simulink model "Ackeraman"  (R2019b)
settings: Solver=VariableStepAuto  StartTime=0.0  StopTime=simTime  RelTol=1e-3
values from neighbouring files (symbols this model uses):
  a0 = 1    [Ackerman_init.m]
  a1 = 4    [Ackerman_init.m]
  a2 = 3    [Ackerman_init.m]
  Change = 0    [Ackerman_init.m]
  k0 = 5    [Ackerman_init.m]
  k1 = place(Ad,bd,pd)    [Ackerman_init.m]
  k2 = place(Ac,bc,lambdatr')    [Ackerman_init.m]
  l = xlabel('Time (s)')    [Ackerman_init.m]
  pathType = 1    [Ackerman_init.m]
  phi0 = 0    [Ackerman_init.m]
  r = 2    [Ackerman_init.m]
  ref0 = [0 0]'    [Ackerman_init.m]
  refType = 1    [Ackerman_init.m]
  T = 0.3    [Ackerman_init.m]
  theta0 = pi    (= 3.14159265359)    [Ackerman_init.m]
  v0 = 2    [Ackerman_init.m]
  v_ref = 2    [Ackerman_init.m]
  x0 = 1    [Ackerman_init.m]
  y0 = 2    [Ackerman_init.m]
libraries: robotmobilelib x4
(part 2 of 4)

== matlab function Ackeraman/MATLAB Function4 ==
  data: state input; v input; v_ref input; c input; pathType parameter; r parameter; a2 parameter; a1 parameter; a0 parameter; k0 parameter; l parameter; u output; w output; Change parameter; T parameter; refType parameter
function [u,w] = MATLAB_Function5(state, v, v_ref, c ,pathType, r, a2, a1, a0, k0, l , Change, T, refType)

x = state(1); y = state(2); z = state(3); theta = state(4);

d = T/3; 
if refType == 1
    L = exp(-k0*T); 
else
    L = 0;  
end
 

if pathType == 1
    w0 = [   -(2*a2*l^2*v^2*cos(theta)^2 - 2*v^3*y*sin(z) - a0*l^2*r^2*cos(theta)^2 - 2*v^3*x*cos(z) + a0*l^2*x^2*cos(theta)^2 + a0*l^2*y^2*cos(theta)^2 + 2*v^3*x*cos(theta)^2*cos(z) + 2*v^3*y*cos(theta)^2*sin(z) + 2*a1*l^2*v*x*cos(theta)^2*cos(z) + 2*a1*l^2*v*y*cos(theta)^2*sin(z) + 2*a2*l*v^2*y*cos(theta)*cos(z)*sin(theta) - 2*a2*l*v^2*x*cos(theta)*sin(theta)*sin(z))/(2*l*v^2*(y*cos(z) - x*sin(z)));
             -(2*a2*l^2*v^2*cos(theta)^2 - 2*v^3*y*sin(z) - a0*l^2*r^2*cos(theta)^2 - 2*v^3*x*cos(z) + a0*l^2*x^2*cos(theta)^2 + a0*l^2*y^2*cos(theta)^2 + 2*v^3*x*cos(theta)^2*cos(z) + 2*v^3*y*cos(theta)^2*sin(z) + 2*a1*l^2*v*x*cos(theta)^2*cos(z) + 2*a1*l^2*v*y*cos(theta)^2*sin(z) + 2*a2*l*v^2*y*cos(theta)*cos(z)*sin(theta) - 2*a2*l*v^2*x*cos(theta)*sin(theta)*sin(z))/(2*l*v^2*(y*cos(z) - x*sin(z)));
             -(2*a2*l^2*v^2*cos(theta)^2 - 2*v^3*y*sin(z) - a0*l^2*r^2*cos(theta)^2 - 2*v^3*x*cos(z) + a0*l^2*x^2*cos(theta)^2 + a0*l^2*y^2*cos(theta)^2 + 2*v^3*x*cos(theta)^2*cos(z) + 2*v^3*y*cos(theta)^2*sin(z) + 2*a1*l^2*v*x*cos(theta)^2*cos(z) + 2*a1*l^2*v*y*cos(theta)^2*sin(z) + 2*a2*l*v^2*y*cos(theta)*cos(z)*sin(theta) - 2*a2*l*v^2*x*cos(theta)*sin(theta)*sin(z))/(2*l*v^2*(y*cos(z) - x*sin(z)))]; 
 
    w1 = [  -(3*(2*l*v^6*y*cos(theta)^3*cos(z) - 2*v^6*y^2*cos(z)^2*sin(theta) - 2*v^6*x^2*sin(theta)*sin(z)^2 - 2*v^6*y^2*sin(theta)*sin(z)^2 - 2*v^6*x^2*cos(z)^2*sin(theta) - 2*l*v^6*x*cos(theta)^3*sin(z) - 2*v^6*x^2*cos(theta)^2*cos(z)^2*sin(theta) + 4*v^6*x^2*cos(theta)^4*cos(z)^2*sin(theta) + 2*v^6*y^2*cos(theta)^2*cos(z)^2*sin(theta) + 2*v^6*x^2*cos(theta)^2*sin(theta)*sin(z)^2 - 2*v^6*y^2*cos(theta)^2*sin(theta)*sin(z)^2 + 4*v^6*y^2*cos(theta)^4*sin(theta)*sin(z)^2 - 2*l*v^6*y*cos(theta)*cos(z) + a0^2*l^4*r^4*cos(theta)^4*sin(theta) + 2*l*v^6*x*cos(theta)*sin(z) + 4*a2^2*l^4*v^4*cos(theta)^4*sin(theta) + a0^2*l^4*x^4*cos(theta)^4*sin(theta) + a0^2*l^4*y^4*cos(theta)^4*sin(theta) - 2*a2^2*l^3*v^4*y*cos(theta)^3*cos(z) + 2*a2^2*l^3*v^4*x*cos(theta)^3*sin(z) - 2*a0^2*l^4*r^2*x^2*cos(theta)^4*sin(theta) - 2*a0^2*l^4*r^2*y^2*cos(theta)^4*sin(theta) + 2*a0^2*l^4*x^2*y^2*cos(theta)^4*sin(theta) + 2*a1*l^3*v^4*y*cos(theta)^3*cos(z) - 2*a1*l^3*v^4*x*cos(theta)^3*sin(z) - 2*a2^2*l^2*v^4*x^2*cos(theta)^2*sin(theta)*sin(z)^2 + 4*a1^2*l^4*v^2*y^2*cos(theta)^4*sin(theta)*sin(z)^2 - 8*v^6*x*y*cos(theta)^2*cos(z)*sin(theta)*sin(z) + 8*v^6*x*y*cos(theta)^4*cos(z)*sin(theta)*sin(z) - a0*l^2*v^3*x^3*cos(theta)^2*cos(z)*sin(theta) + 4*a0*l^2*v^3*x^3*cos(theta)^4*cos(z)*sin(theta) - 2*a0*l^3*v^3*x^2*cos(theta)^3*cos(z)*sin(z) + 2*a0*l^3*v^3*y^2*cos(theta)^3*cos(z)*sin(z) - a0*l^2*v^3*y^3*cos(theta)^2*sin(theta)*sin(z) + 4*a0*l^2*v^3*y^3*cos(theta)^4*sin(theta)*sin(z) + 4*a2^2*l^2*v^4*y^2*cos(theta)^2*cos(z)^2*sin(theta)^3 + 4*a2^2*l^2*v^4*x^2*cos(theta)^2*sin(theta)^3*sin(z)^2 - 2*a1*l^2*v^4*x^2*cos(theta)^2*cos(z)^2*sin(theta) + 8*a1*l^2*v^4*x^2*cos(theta)^4*cos(z)^2*sin(theta) + 2*a1*l^2*v^4*y^2*cos(theta)^2*cos(z)^2*sin(theta) + 8*a2^2*l^3*v^4*y*cos(theta)^3*cos(z)*sin(theta)^2 + 2*a1*l^2*v^4*x^2*cos(theta)^2*sin(theta)*sin(z)^2 - 8*a2^2*l^3*v^4*x*cos(theta)^3*sin(theta)^2*sin(z) - 2*a1*l^2*v^4*y^2*cos(theta)^2*sin(theta)*sin(z)^2 + 8*a1*l^2*v^4*y^2*cos(theta)^4*sin(theta)*sin(z)^2 - a0*a2*l^3*v^2*y^3*cos(theta)^3*cos(z) - 4*a0*a2*l^4*r^2*v^2*cos(theta)^4*sin(theta) + 4*a0*a2*l^4*v^2*x^2*cos(theta)^4*sin(theta) + 4*a0*a2*l^4*v^2*y^2*cos(theta)^4*sin(theta) + a0*a2*l^3*v^2*x^3*cos(theta)^3*sin(z) + 2*a0*l^3*v^3*x*y*cos(theta)^3*cos(z)^2 - 2*a2*l^2*v^5*x*cos(theta)^2*cos(z)*sin(theta) + 8*a2*l^2*v^5*x*cos(theta)^4*cos(z)*sin(theta) - 2*a0*l^3*v^3*x*y*cos(theta)^3*sin(z)^2 - 2*a2*l^2*v^5*y*cos(theta)^2*sin(theta)*sin(z) + 8*a2*l^2*v^5*y*cos(theta)^4*sin(theta)*sin(z) + 4*a1^2*l^4*v^2*x^2*cos(theta)^4*cos(z)^2*sin(theta) - 2*a2^2*l^2*v^4*y^2*cos(theta)^2*cos(z)^2*sin(theta) - 4*a0*a2*l^3*v^2*x^3*cos(theta)^3*sin(theta)^2*sin(z) + a0*a2*l^3*r^2*v^2*y*cos(theta)^3*cos(z) - 8*a2*l*v^5*x^2*cos(theta)^3*cos(z)*sin(theta)^2*sin(z) + 8*a2*l*v^5*y^2*cos(theta)^3*cos(z)*sin(theta)^2*sin(z) - a0*a2*l^3*v^2*x^2*y*cos(theta)^3*cos(z) - 2*a1*a2*l^3*v^3*x*y*cos(theta)^3*cos(z)^2 - a0*a2*l^3*r^2*v^2*x*cos(theta)^3*sin(z) + 4*a0*a1*l^4*v*x^3*cos(theta)^4*cos(z)*sin(theta) + 8*a1*a2*l^4*v^3*x*cos(theta)^4*cos(z)*sin(theta) + a0*a2*l^3*v^2*x*y^2*cos(theta)^3*sin(z) + 2*a1*a2*l^3*v^3*x*y*cos(theta)^3*sin(z)^2 + 4*a0*a1*l^4*v*y^3*cos(theta)^4*sin(theta)*sin(z) + 8*a1*a2*l^4*v^3*y*cos(theta)^4*sin(theta)*sin(z) - 2*a2*l*v^5*x*y*cos(theta)*cos(z)^2*sin(theta)^2 + 2*a2*l*v^5*x*y*cos(theta)*sin(theta)^2*sin(z)^2 + 2*a1*a2*l^3*v^3*x^2*cos(theta)^3*cos(z)*sin(z) - 2*a1*a2*l^3*v^3*y^2*cos(theta)^3*cos(z)*sin(z) + a0*l^2*r^2*v^3*x*cos(theta)^2*cos(z)*sin(theta) - 4*a0*l^2*r^2*v^3*x*cos(theta)^4*cos(z)*sin(theta) - a0*l^2*v^3*x*y^2*cos(theta)^2*cos(z)*sin(theta) + 4*a0*l^2*v^3*x*y^2*cos(theta)^4*cos(z)*sin(theta) + 8*a2*l*v^5*x*y*cos(theta)^3*cos(z)^2*sin(theta)^2 + a0*l^2*r^2*v^3*y*cos(theta)^2*sin(theta)*sin(z) - 4*a0*l^2*r^2*v^3*y*cos(theta)^4*sin(theta)*sin(z) - a0*l^2*v^3*x^2*y*cos(theta)^2*sin(theta)*sin(z) + 4*a0*l^2*v^3*x^2*y*cos(theta)^4*sin(theta)*sin(z) - 8*a2*l*v^5*x*y*cos(theta)^3*sin(theta)^2*sin(z)^2 + 2*a2*l*v^5*x^2*cos(theta)*cos(z)*sin(theta)^2*sin(z) - 2*a2*l*v^5*y^2*cos(theta)*cos(z)*sin(theta)^2*sin(z) + 4*a0*a2*l^3*v^2*y^3*cos(theta)^3*cos(z)*sin(theta)^2 - 8*a1*l^2*v^4*x*y*cos(theta)^2*cos(z)*sin(theta)*sin(z) + 16*a1*l^2*v^4*x*y*cos(theta)^4*cos(z)*sin(theta)*sin(z) - 4*a0*a2*l^3*r^2*v^2*y*cos(theta)^3*cos(z)*sin(theta)^2 + 4*a0*a2*l^3*v^2*x^2*y*cos(theta)^3*cos(z)*sin(theta)^2 + 8*a1*a2*l^3*v^3*x*y*cos(theta)^3*cos(z)^2*sin(theta)^2 + 4*a0*a2*l^3*r^2*v^2*x*cos(theta)^3*sin(theta)^2*sin(z) - 4*a0*a2*l^3*v^2*x*y^2*cos(theta)^3*sin(theta)^2*sin(z) - 8*a1*a2*l^3*v^3*x*y*cos(theta)^3*sin(theta)^2*sin(z)^2 + 4*a2^2*l^2*v^4*x*y*cos(theta)^2*cos(z)*sin(theta)*sin(z) + 8*a1^2*l^4*v^2*x*y*cos(theta)^4*cos(z)*sin(theta)*sin(z) - 4*a0*a1*l^4*r^2*v*x*cos(theta)^4*cos(z)*sin(theta) + 4*a0*a1*l^4*v*x*y^2*cos(theta)^4*cos(z)*sin(theta) - 4*a0*a1*l^4*r^2*v*y*cos(theta)^4*sin(theta)*sin(z) + 4*a0*a1*l^4*v*x^2*y*cos(theta)^4*sin(theta)*sin(z) - 8*a1*a2*l^3*v^3*x^2*cos(theta)^3*cos(z)*sin(theta)^2*sin(z) + 8*a1*a2*l^3*v^3*y^2*cos(theta)^3*cos(z)*sin(theta)^2*sin(z) - 8*a2^2*l^2*v^4*x*y*cos(theta)^2*cos(z)*sin(theta)^3*sin(z)))/(8*l^2*v^4*cos(theta)*(y*cos(z) - x*sin(z))^2);
            -(3*(2*l*v^6*y*cos(theta)^3*cos(z) - 2*v^6*y^2*cos(z)^2*sin(theta) - 2*v^6*x^2*sin(theta)*sin(z)^2 - 2*v^6*y^2*sin(theta)*sin(z)^2 - 2*v^6*x^2*cos(z)^2*sin(theta) - 2*l*v^6*x*cos(theta)^3*sin(z) - 2*v^6*x^2*cos(theta)^2*cos(z)^2*sin(theta) + 4*v^6*x^2*cos(theta)^4*cos(z)^2*sin(theta) + 2*v^6*y^2*cos(theta)^2*cos(z)^2*sin(theta) + 2*v^6*x^2*cos(theta)^2*sin(theta)*sin(z)^2 - 2*v^6*y^2*cos(theta)^2*sin(theta)*sin(z)^2 + 4*v^6*y^2*cos(theta)^4*sin(theta)*sin(z)^2 - 2*l*v^6*y*cos(theta)*cos(z) + a0^2*l^4*r^4*cos(theta)^4*sin(theta) + 2*l*v^6*x*cos(theta)*sin(z) + 4*a2^2*l^4*v^4*cos(theta)^4*sin(theta) + a0^2*l^4*x^4*cos(theta)^4*sin(theta) + a0^2*l^4*y^4*cos(theta)^4*sin(theta) - 2*a2^2*l^3*v^4*y*cos(theta)^3*cos(z) + 2*a2^2*l^3*v^4*x*cos(theta)^3*sin(z) - 2*a0^2*l^4*r^2*x^2*cos(theta)^4*sin(theta) - 2*a0^2*l^4*r^2*y^2*cos(theta)^4*sin(theta) + 2*a0^2*l^4*x^2*y^2*cos(theta)^4*sin(theta) + 2*a1*l^3*v^4*y*cos(theta)^3*cos(z) - 2*a1*l^3*v^4*x*cos(theta)^3*sin(z) - 2*a2^2*l^2*v^4*x^2*cos(theta)^2*sin(theta)*sin(z)^2 + 4*a1^2*l^4*v^2*y^2*cos(theta)^4*sin(theta)*sin(z)^2 - 8*v^6*x*y*cos(theta)^2*cos(z)*sin(theta)*sin(z) + 8*v^6*x*y*cos(theta)^4*cos(z)*sin(theta)*sin(z) - a0*l^2*v^3*x^3*cos(theta)^2*cos(z)*sin(theta) + 4*a0*l^2*v^3*x^3*cos(theta)^4*cos(z)*sin(theta) - 2*a0*l^3*v^3*x^2*cos(theta)^3*cos(z)*sin(z) + 2*a0*l^3*v^3*y^2*cos(theta)^3*cos(z)*sin(z) - a0*l^2*v^3*y^3*cos(theta)^2*sin(theta)*sin(z) + 4*a0*l^2*v^3*y^3*cos(theta)^4*sin(theta)*sin(z) + 4*a2^2*l^2*v^4*y^2*cos(theta)^2*cos(z)^2*sin(theta)^3 + 4*a2^2*l^2*v^4*x^2*cos(theta)^2*sin(theta)^3*sin(z)^2 - 2*a1*l^2*v^4*x^2*cos(theta)^2*cos(z)^2*sin(theta) + 8*a1*l^2*v^4*x^2*cos(theta)^4*cos(z)^2*sin(theta) + 2*a1*l^2*v^4*y^2*cos(theta)^2*cos(z)^2*sin(theta) + 8*a2^2*l^3*v^4*y*cos(theta)^3*cos(z)*sin(theta)^2 + 2*a1*l^2*v^4*x^2*cos(theta)^2*sin(theta)*sin(z)^2 - 8*a2^2*l^3*v^4*x*cos(theta)^3*sin(theta)^2*sin(z) - 2*a1*l^2*v^4*y^2*cos(theta)^2*sin(theta)*sin(z)^2 + 8*a1*l^2*v^4*y^2*cos(theta)^4*sin(theta)*sin(z)^2 - a0*a2*l^3*v^2*y^3*cos(theta)^3*cos(z) - 4*a0*a2*l^4*r^2*v^2*cos(theta)^4*sin(theta) + 4*a0*a2*l^4*v^2*x^2*cos(theta)^4*sin(theta) + 4*a0*a2*l^4*v^2*y^2*cos(theta)^4*sin(theta) + a0*a2*l^3*v^2*x^3*cos(theta)^3*sin(z) + 2*a0*l^3*v^3*x*y*cos(theta)^3*cos(z)^2 - 2*a2*l^2*v^5*x*cos(theta)^2*cos(z)*sin(theta) + 8*a2*l^2*v^5*x*cos(theta)^4*cos(z)*sin(theta) - 2*a0*l^3*v^3*x*y*cos(theta)^3*sin(z)^2 - 2*a2*l^2*v^5*y*cos(theta)^2*sin(theta)*sin(z) + 8*a2*l^2*v^5*y*cos(theta)^4*sin(theta)*sin(z) + 4*a1^2*l^4*v^2*x^2*cos(theta)^4*cos(z)^2*sin(theta) - 2*a2^2*l^2*v^4*y^2*cos(theta)^2*cos(z)^2*sin(theta) - 4*a0*a2*l^3*v^2*x^3*cos(theta)^3*sin(theta)^2*sin(z) + a0*a2*l^3*r^2*v^2*y*cos(theta)^3*cos(z) - 8*a2*l*v^5*x^2*cos(theta)^3*cos(z)*sin(theta)^2*sin(z) + 8*a2*l*v^5*y^2*cos(theta)^3*cos(z)*sin(theta)^2*sin(z) - a0*a2*l^3*v^2*x^2*y*cos(theta)^3*cos(z) - 2*a1*a2*l^3*v^3*x*y*cos(theta)^3*cos(z)^2 - a0*a2*l^3*r^2*v^2*x*cos(theta)^3*sin(z) + 4*a0*a1*l^4*v*x^3*cos(theta)^4*cos(z)*sin(theta) + 8*a1*a2*l^4*v^3*x*cos(theta)^4*cos(z)*sin(theta) + a0*a2*l^3*v^2*x*y^2*cos(theta)^3*sin(z) + 2*a1*a2*l^3*v^3*x*y*cos(theta)^3*sin(z)^2 + 4*a0*a1*l^4*v*y^3*cos(theta)^4*sin(theta)*sin(z) + 8*a1*a2*l^4*v^3*y*cos(theta)^4*sin(theta)*sin(z) - 2*a2*l*v^5*x*y*cos(theta)*cos(z)^2*sin(theta)^2 + 2*a2*l*v^5*x*y*cos(theta)*sin(theta)^2*sin(z)^2 + 2*a1*a2*l^3*v^3*x^2*cos(theta)^3*cos(z)*sin(z) - 2*a1*a2*l^3*v^3*y^2*cos(theta)^3*cos(z)*sin(z) + a0*l^2*r^2*v^3*x*cos(theta)^2*cos(z)*sin(theta) - 4*a0*l^2*r^2*v^3*x*cos(theta)^4*cos(z)*sin(theta) - a0*l^2*v^3*x*y^2*cos(theta)^2*cos(z)*sin(theta) + 4*a0*l^2*v^3*x*y^2*cos(theta)^4*cos(z)*sin(theta) + 8*a2*l*v^5*x*y*cos(theta)^3*cos(z)^2*sin(theta)^2 + a0*l^2*r^2*v^3*y*cos(theta)^2*sin(theta)*sin(z) - 4*a0*l^2*r^2*v^3*y*cos(theta)^4*sin(theta)*sin(z) - a0*l^2*v^3*x^2*y*cos(theta)^2*sin(theta)*sin(z) + 4*a0*l^2*v^3*x^2*y*cos(theta)^4*sin(theta)*sin(z) - 8*a2*l*v^5*x*y*cos(theta)^3*sin(theta)^2*sin(z)^2 + 2*a2*l*v^5*x^2*cos(theta)*cos(z)*sin(theta)^2*sin(z) - 2*a2*l*v^5*y^2*cos(theta)*cos(z)*sin(theta)^2*sin(z) + 4*a0*a2*l^3*v^2*y^3*cos(theta)^3*cos(z)*sin(theta)^2 - 8*a1*l^2*v^4*x*y*cos(theta)^2*cos(z)*sin(theta)*sin(z) + 16*a1*l^2*v^4*x*y*cos(theta)^4*cos(z)*sin(theta)*sin(z) - 4*a0*a2*l^3*r^2*v^2*y*cos(theta)^3*cos(z)*sin(theta)^2 + 4*a0*a2*l^3*v^2*x^2*y*cos(theta)^3*cos(z)*sin(theta)^2 + 8*a1*a2*l^3*v^3*x*y*cos(theta)^3*cos(z)^2*sin(theta)^2 + 4*a0*a2*l^3*r^2*v^2*x*cos(theta)^3*sin(theta)^2*sin(z) - 4*a0*a2*l^3*v^2*x*y^2*cos(theta)^3*sin(theta)^2*sin(z) - 8*a1*a2*l^3*v^3*x*y*cos(theta)^3*sin(theta)^2*sin(z)^2 + 4*a2^2*l^2*v^4*x*y*cos(theta)^2*cos(z)*sin(theta)*sin(z) + 8*a1^2*l^4*v^2*x*y*cos(theta)^4*cos(z)*sin(theta)*sin(z) - 4*a0*a1*l^4*r^2*v*x*cos(theta)^4*cos(z)*sin(theta) + 4*a0*a1*l^4*v*x*y^2*cos(theta)^4*cos(z)*sin(theta) - 4*a0*a1*l^4*r^2*v*y*cos(theta)^4*sin(theta)*sin(z) + 4*a0*a1*l^4*v*x^2*y*cos(theta)^4*sin(theta)*sin(z) - 8*a1*a2*l^3*v^3*x^2*cos(theta)^3*cos(z)*sin(theta)^2*sin(z) + 8*a1*a2*l^3*v^3*y^2*cos(theta)^3*cos(z)*sin(theta)^2*sin(z) - 8*a2^2*l^2*v^4*x*y*cos(theta)^2*cos(z)*sin(theta)^3*sin(z)))/(2*l^2*v^4*cos(theta)*(y*cos(z) - x*sin(z))^2);
            -(21*(2*l*v^6*y*cos(theta)^3*cos(z) - 2*v^6*y^2*cos(z)^2*sin(theta) - 2*v^6*x^2*sin(theta)*sin(z)^2 - 2*v^6*y^2*sin(theta)*sin(z)^2 - 2*v^6*x^2*cos(z)^2*sin(theta) - 2*l*v^6*x*cos(theta)^3*sin(z) - 2*v^6*x^2*cos(theta)^2*cos(z)^2*sin(theta) + 4*v^6*x^2*cos(theta)^4*cos(z)^2*sin(theta) + 2*v^6*y^2*cos(theta)^2*cos(z)^2*sin(theta) + 2*v^6*x^2*cos(theta)^2*sin(theta)*sin(z)^2 - 2*v^6*y^2*cos(theta)^2*sin(theta)*sin(z)^2 + 4*v^6*y^2*cos(theta)^4*sin(theta)*sin(z)^2 - 2*l*v^6*y*cos(theta)*cos(z) + a0^2*l^4*r^4*cos(theta)^4*sin(theta) + 2*l*v^6*x*cos(theta)*sin(z) + 4*a2^2*l^4*v^4*cos(theta)^4*sin(theta) + a0^2*l^4*x^4*cos(theta)^4*sin(theta) + a0^2*l^4*y^4*cos(theta)^4*sin(theta) - 2*a2^2*l^3*v^4*y*cos(theta)^3*cos(z) + 2*a2^2*l^3*v^4*x*cos(theta)^3*sin(z) - 2*a0^2*l^4*r^2*x^2*cos(theta)^4*sin(theta) - 2*a0^2*l^4*r^2*y^2*cos(theta)^4*sin(theta) + 2*a0^2*l^4*x^2*y^2*cos(theta)^4*sin(theta) + 2*a1*l^3*v^4*y*cos(theta)^3*cos(z) - 2*a1*l^3*v^4*x*cos(theta)^3*sin(z) - 2*a2^2*l^2*v^4*x^2*cos(theta)^2*sin(theta)*sin(z)^2 + 4*a1^2*l^4*v^2*y^2*cos(theta)^4*sin(theta)*sin(z)^2 - 8*v^6*x*y*cos(theta)^2*cos(z)*sin(theta)*sin(z) + 8*v^6*x*y*cos(theta)^4*cos(z)*sin(theta)*sin(z) - a0*l^2*v^3*x^3*cos(theta)^2*cos(z)*sin(theta) + 4*a0*l^2*v^3*x^3*cos(theta)^4*cos(z)*sin(theta) - 2*a0*l^3*v^3*x^2*cos(theta)^3*cos(z)*sin(z) + 2*a0*l^3*v^3*y^2*cos(theta)^3*cos(z)*sin(z) - a0*l^2*v^3*y^3*cos(theta)^2*sin(theta)*sin(z) + 4*a0*l^2*v^3*y^3*cos(theta)^4*sin(theta)*sin(z) + 4*a2^2*l^2*v^4*y^2*cos(theta)^2*cos(z)^2*sin(theta)^3 + 4*a2^2*l^2*v^4*x^2*cos(theta)^2*sin(theta)^3*sin(z)^2 - 2*a1*l^2*v^4*x^2*cos(theta)^2*cos(z)^2*sin(theta) + 8*a1*l^2*v^4*x^2*cos(theta)^4*cos(z)^2*sin(theta) + 2*a1*l^2*v^4*y^2*cos(theta)^2*cos(z)^2*sin(theta) + 8*a2^2*l^3*v^4*y*cos(theta)^3*cos(z)*sin(theta)^2 + 2*a1*l^2*v^4*x^2*cos(theta)^2*sin(theta)*sin(z)^2 - 8*a2^2*l^3*v^4*x*cos(theta)^3*sin(theta)^2*sin(z) - 2*a1*l^2*v^4*y^2*cos(theta)^2*sin(theta)*sin(z)^2 + 8*a1*l^2*v^4*y^2*cos(theta)^4*sin(theta)*sin(z)^2 - a0*a2*l^3*v^2*y^3*cos(theta)^3*cos(z) - 4*a0*a2*l^4*r^2*v^2*cos(theta)^4*sin(theta) + 4*a0*a2*l^4*v^2*x^2*cos(theta)^4*sin(theta) + 4*a0*a2*l^4*v^2*y^2*cos(theta)^4*sin(theta) + a0*a2*l^3*v^2*x^3*cos(theta)^3*sin(z) + 2*a0*l^3*v^3*x*y*cos(theta)^3*cos(z)^2 - 2*a2*l^2*v^5*x*cos(theta)^2*cos(z)*sin(theta) + 8*a2*l^2*v^5*x*cos(theta)^4*cos(z)*sin(theta) - 2*a0*l^3*v^3*x*y*cos(theta)^3*sin(z)^2 - 2*a2*l^2*v^5*y*cos(theta)^2*sin(theta)*sin(z) + 8*a2*l^2*v^5*y*cos(theta)^4*sin(theta)*sin(z) + 4*a1^2*l^4*v^2*x^2*cos(theta)^4*cos(z)^2*sin(theta) - 2*a2^2*l^2*v^4*y^2*cos(theta)^2*cos(z)^2*sin(theta) - 4*a0*a2*l^3*v^2*x^3*cos(theta)^3*sin(theta)^2*sin(z) + a0*a2*l^3*r^2*v^2*y*cos(theta)^3*cos(z) - 8*a2*l*v^5*x^2*cos(theta)^3*cos(z)*sin(theta)^2*sin(z) + 8*a2*l*v^5*y^2*cos(theta)^3*cos(z)*sin(theta)^2*sin(z) - a0*a2*l^3*v^2*x^2*y*cos(theta)^3*cos(z) - 2*a1*a2*l^3*v^3*x*y*cos(theta)^3*cos(z)^2 - a0*a2*l^3*r^2*v^2*x*cos(theta)^3*sin(z) + 4*a0*a1*l^4*v*x^3*cos(theta)^4*cos(z)*sin(theta) + 8*a1*a2*l^4*v^3*x*cos(theta)^4*cos(z)*sin(theta) + a0*a2*l^3*v^2*x*y^2*cos(theta)^3*sin(z) + 2*a1*a2*l^3*v^3*x*y*cos(theta)^3*sin(z)^2 + 4*a0*a1*l^4*v*y^3*cos(theta)^4*sin(theta)*sin(z) + 8*a1*a2*l^4*v^3*y*cos(theta)^4*sin(theta)*sin(z) - 2*a2*l*v^5*x*y*cos(theta)*cos(z)^2*sin(theta)^2 + 2*a2*l*v^5*x*y*cos(theta)*sin(theta)^2*sin(z)^2 + 2*a1*a2*l^3*v^3*x^2*cos(theta)^3*cos(z)*sin(z) - 2*a1*a2*l^3*v^3*y^2*cos(theta)^3*cos(z)*sin(z) + a0*l^2*r^2*v^3*x*cos(theta)^2*cos(z)*sin(theta) - 4*a0*l^2*r^2*v^3*x*cos(theta)^4*cos(z)*sin(theta) - a0*l^2*v^3*x*y^2*cos(theta)^2*cos(z)*sin(theta) + 4*a0*l^2*v^3*x*y^2*cos(theta)^4*cos(z)*sin(theta) + 8*a2*l*v^5*x*y*cos(theta)^3*cos(z)^2*sin(theta)^2 + a0*l^2*r^2*v^3*y*cos(theta)^2*sin(theta)*sin(z) - 4*a0*l^2*r^2*v^3*y*cos(theta)^4*sin(theta)*sin(z) - a0*l^2*v^3*x^2*y*cos(theta)^2*sin(theta)*sin(z) + 4*a0*l^2*v^3*x^2*y*cos(theta)^4*sin(theta)*sin(z) - 8*a2*l*v^5*x*y*cos(theta)^3*sin(theta)^2*sin(z)^2 + 2*a2*l*v^5*x^2*cos(theta)*cos(z)*sin(theta)^2*sin(z) - 2*a2*l*v^5*y^2*cos(theta)*cos(z)*sin(theta)^2*sin(z) + 4*a0*a2*l^3*v^2*y^3*cos(theta)^3*cos(z)*sin(theta)^2 - 8*a1*l^2*v^4*x*y*cos(theta)^2*cos(z)*sin(theta)*sin(z) + 16*a1*l^2*v^4*x*y*cos(theta)^4*cos(z)*sin(theta)*sin(z) - 4*a0*a2*l^3*r^2*v^2*y*cos(theta)^3*cos(z)*sin(theta)^2 + 4*a0*a2*l^3*v^2*x^2*y*cos(theta)^3*cos(z)*sin(theta)^2 + 8*a1*a2*l^3*v^3*x*y*cos(theta)^3*cos(z)^2*sin(theta)^2 + 4*a0*a2*l^3*r^2*v^2*x*cos(theta)^3*sin(theta)^2*sin(z) - 4*a0*a2*l^3*v^2*x*y^2*cos(theta)^3*sin(theta)^2*sin(z) - 8*a1*a2*l^3*v^3*x*y*cos(theta)^3*sin(theta)^2*sin(z)^2 + 4*a2^2*l^2*v^4*x*y*cos(theta)^2*cos(z)*sin(theta)*sin(z) + 8*a1^2*l^4*v^2*x*y*cos(theta)^4*cos(z)*sin(theta)*sin(z) - 4*a0*a1*l^4*r^2*v*x*cos(theta)^4*cos(z)*sin(theta) + 4*a0*a1*l^4*v*x*y^2*cos(theta)^4*cos(z)*sin(theta) - 4*a0*a1*l^4*r^2*v*y*cos(theta)^4*sin(theta)*sin(z) + 4*a0*a1*l^4*v*x^2*y*cos(theta)^4*sin(theta)*sin(z) - 8*a1*a2*l^3*v^3*x^2*cos(theta)^3*cos(z)*sin(theta)^2*sin(z) + 8*a1*a2*l^3*v^3*y^2*cos(theta)^3*cos(z)*sin(theta)^2*sin(z) - 8*a2^2*l^2*v^4*x*y*cos(theta)^2*cos(z)*sin(theta)^3*sin(z)))/(8*l^2*v^4*cos(theta)*(y*cos(z) - x*sin(z))^2)];

else
    
       w0 = [-(2533274790395904*v^3*x*cos(z) - 2533274790395904*v^3*y*sin(z) - 1228357238169957*a0*l^2*cos(theta)^2 - 281474976710656*v^3*x^3*cos(z) - 281474976710656*v^3*y^3*sin(z) + 281474976710656*v^3*x^3*cos(theta)^2*cos(z) + 281474976710656*v^3*y^3*cos(theta)^2*sin(z) - 281474976710656*v^3*x*y^2*cos(z) - 281474976710656*v^3*x^2*y*sin(z) + 2533274790395904*a2*l^2*v^2*cos(theta)^2 - 1266637395197952*a0*l^2*x^2*cos(theta)^2 + 70368744177664*a0*l^2*x^4*cos(theta)^2 + 1266637395197952*a0*l^2*y^2*cos(theta)^2 + 70368744177664*a0*l^2*y^4*cos(theta)^2 - 2533274790395904*v^3*x*cos(theta)^2*cos(z) + 2533274790395904*v^3*y*cos(theta)^2*sin(z) + 281474976710656*a2*l^2*v^2*x^2*cos(theta)^2 + 844424930131968*a2*l^2*v^2*y^2*cos(theta)^2 + 140737488355328*a0*l^2*x^2*y^2*cos(theta)^2 + 1688849860263936*l^2*v^3*x*cos(theta)^2*cos(z) + 281474976710656*v^3*x*y^2*cos(theta)^2*cos(z) + 1688849860263936*l^2*v^3*y*cos(theta)^2*sin(z) + 281474976710656*v^3*x^2*y*cos(theta)^2*sin(z) - 5066549580791808*a2*l^2*v^2*cos(theta)^2*cos(z)^2 - 844424930131968*l*v^3*x*y*sin(2*theta) + 15199648742375424*l*v^3*cos(theta)*cos(z)*sin(theta)*sin(z) - 2533274790395904*a1*l^2*v*x*cos(theta)^2*cos(z) + 2533274790395904*a1*l^2*v*y*cos(theta)^2*sin(z) + 562949953421312*a2*l^2*v^2*x^2*cos(theta)^2*cos(z)^2 - 562949953421312*a2*l^2*v^2*y^2*cos(theta)^2*cos(z)^2 + 281474976710656*a1*l^2*v*x^3*cos(theta)^2*cos(z) + 281474976710656*a1*l^2*v*y^3*cos(theta)^2*sin(z) - 1688849860263936*l*v^3*x^2*cos(theta)*cos(z)*sin(theta)*sin(z) + 1688849860263936*l*v^3*y^2*cos(theta)*cos(z)*sin(theta)*sin(z) + 2533274790395904*a2*l*v^2*y*cos(theta)*cos(z)*sin(theta) + 2533274790395904*a2*l*v^2*x*cos(theta)*sin(theta)*sin(z) + 281474976710656*a1*l^2*v*x*y^2*cos(theta)^2*cos(z) + 281474976710656*a1*l^2*v*x^2*y*cos(theta)^2*sin(z) + 281474976710656*a2*l*v^2*y^3*cos(theta)*cos(z)*sin(theta) - 281474976710656*a2*l*v^2*x^3*cos(theta)*sin(theta)*sin(z) + 3377699720527872*l*v^3*x*y*cos(theta)*cos(z)^2*sin(theta) + 1125899906842624*a2*l^2*v^2*x*y*cos(theta)^2*cos(z)*sin(z) + 281474976710656*a2*l*v^2*x^2*y*cos(theta)*cos(z)*sin(theta) - 281474976710656*a2*l*v^2*x*y^2*cos(theta)*sin(theta)*sin(z))/(281474976710656*l*v^2*(- sin(z)*x^3 + cos(z)*x^2*y - sin(z)*x*y^2 + 9*sin(z)*x + cos(z)*y^3 + 9*cos(z)*y));
        -(2533274790395904*v^3*x*cos(z) - 2533274790395904*v^3*y*sin(z) - 1228357238169957*a0*l^2*cos(theta)^2 - 281474976710656*v^3*x^3*cos(z) - 281474976710656*v^3*y^3*sin(z) + 281474976710656*v^3*x^3*cos(theta)^2*cos(z) + 281474976710656*v^3*y^3*cos(theta)^2*sin(z) - 281474976710656*v^3*x*y^2*cos(z) - 281474976710656*v^3*x^2*y*sin(z) + 2533274790395904*a2*l^2*v^2*cos(theta)^2 - 1266637395197952*a0*l^2*x^2*cos(theta)^2 + 70368744177664*a0*l^2*x^4*cos(theta)^2 + 1266637395197952*a0*l^2*y^2*cos(theta)^2 + 70368744177664*a0*l^2*y^4*cos(theta)^2 - 2533274790395904*v^3*x*cos(theta)^2*cos(z) + 2533274790395904*v^3*y*cos(theta)^2*sin(z) + 281474976710656*a2*l^2*v^2*x^2*cos(theta)^2 + 844424930131968*a2*l^2*v^2*y^2*cos(theta)^2 + 140737488355328*a0*l^2*x^2*y^2*cos(theta)^2 + 1688849860263936*l^2*v^3*x*cos(theta)^2*cos(z) + 281474976710656*v^3*x*y^2*cos(theta)^2*cos(z) + 1688849860263936*l^2*v^3*y*cos(theta)^2*sin(z) + 281474976710656*v^3*x^2*y*cos(theta)^2*sin(z) - 5066549580791808*a2*l^2*v^2*cos(theta)^2*cos(z)^2 - 844424930131968*l*v^3*x*y*sin(2*theta) + 15199648742375424*l*v^3*cos(theta)*cos(z)*sin(theta)*sin(z) - 2533274790395904*a1*l^2*v*x*cos(theta)^2*cos(z) + 2533274790395904*a1*l^2*v*y*cos(theta)^2*sin(z) + 562949953421312*a2*l^2*v^2*x^2*cos(theta)^2*cos(z)^2 - 562949953421312*a2*l^2*v^2*y^2*cos(theta)^2*cos(z)^2 + 281474976710656*a1*l^2*v*x^3*cos(theta)^2*cos(z) + 281474976710656*a1*l^2*v*y^3*cos(theta)^2*sin(z) - 1688849860263936*l*v^3*x^2*cos(theta)*cos(z)*sin(theta)*sin(z) + 1688849860263936*l*v^3*y^2*cos(theta)*cos(z)*sin(theta)*sin(z) + 2533274790395904*a2*l*v^2*y*cos(theta)*cos(z)*sin(theta) + 2533274790395904*a2*l*v^2*x*cos(theta)*sin(theta)*sin(z) + 281474976710656*a1*l^2*v*x*y^2*cos(theta)^2*cos(z) + 281474976710656*a1*l^2*v*x^2*y*cos(theta)^2*sin(z) + 281474976710656*a2*l*v^2*y^3*cos(theta)*cos(z)*sin(theta) - 281474976710656*a2*l*v^2*x^3*cos(theta)*sin(theta)*sin(z) + 3377699720527872*l*v^3*x*y*cos(theta)*cos(z)^2*sin(theta) + 1125899906842624*a2*l^2*v^2*x*y*cos(theta)^2*cos(z)*sin(z) + 281474976710656*a2*l*v^2*x^2*y*cos(theta)*cos(z)*sin(theta) - 281474976710656*a2*l*v^2*x*y^2*cos(theta)*sin(theta)*sin(z))/(281474976710656*l*v^2*(- sin(z)*x^3 + cos(z)*x^2*y - sin(z)*x*y^2 + 9*sin(z)*x + cos(z)*y^3 + 9*cos(z)*y));
        -(2533274790395904*v^3*x*cos(z) - 2533274790395904*v^3*y*sin(z) - 1228357238169957*a0*l^2*cos(theta)^2 - 281474976710656*v^3*x^3*cos(z) - 281474976710656*v^3*y^3*sin(z) + 281474976710656*v^3*x^3*cos(theta)^2*cos(z) + 281474976710656*v^3*y^3*cos(theta)^2*sin(z) - 281474976710656*v^3*x*y^2*cos(z) - 281474976710656*v^3*x^2*y*sin(z) + 2533274790395904*a2*l^2*v^2*cos(theta)^2 - 1266637395197952*a0*l^2*x^2*cos(theta)^2 + 70368744177664*a0*l^2*x^4*cos(theta)^2 + 1266637395197952*a0*l^2*y^2*cos(theta)^2 + 70368744177664*a0*l^2*y^4*cos(theta)^2 - 2533274790395904*v^3*x*cos(theta)^2*cos(z) + 2533274790395904*v^3*y*cos(theta)^2*sin(z) + 281474976710656*a2*l^2*v^2*x^2*cos(theta)^2 + 844424930131968*a2*l^2*v^2*y^2*cos(theta)^2 + 140737488355328*a0*l^2*x^2*y^2*cos(theta)^2 + 1688849860263936*l^2*v^3*x*cos(theta)^2*cos(z) + 281474976710656*v^3*x*y^2*cos(theta)^2*cos(z) + 1688849860263936*l^2*v^3*y*cos(theta)^2*sin(z) + 281474976710656*v^3*x^2*y*cos(theta)^2*sin(z) - 5066549580791808*a2*l^2*v^2*cos(theta)^2*cos(z)^2 - 844424930131968*l*v^3*x*y*sin(2*theta) + 15199648742375424*l*v^3*cos(theta)*cos(z)*sin(theta)*sin(z) - 2533274790395904*a1*l^2*v*x*cos(theta)^2*cos(z) + 2533274790395904*a1*l^2*v*y*cos(theta)^2*sin(z) + 562949953421312*a2*l^2*v^2*x^2*cos(theta)^2*cos(z)^2 - 562949953421312*a2*l^2*v^2*y^2*cos(theta)^2*cos(z)^2 + 281474976710656*a1*l^2*v*x^3*cos(theta)^2*cos(z) + 281474976710656*a1*l^2*v*y^3*cos(theta)^2*sin(z) - 1688849860263936*l*v^3*x^2*cos(theta)*cos(z)*sin(theta)*sin(z) + 1688849860263936*l*v^3*y^2*cos(theta)*cos(z)*sin(theta)*sin(z) + 2533274790395904*a2*l*v^2*y*cos(theta)*cos(z)*sin(theta) + 2533274790395904*a2*l*v^2*x*cos(theta)*sin(theta)*sin(z) + 281474976710656*a1*l^2*v*x*y^2*cos(theta)^2*cos(z) + 281474976710656*a1*l^2*v*x^2*y*cos(theta)^2*sin(z) + 281474976710656*a2*l*v^2*y^3*cos(theta)*cos(z)*sin(theta) - 281474976710656*a2*l*v^2*x^3*cos(theta)*sin(theta)*sin(z) + 3377699720527872*l*v^3*x*y*cos(theta)*cos(z)^2*sin(theta) + 1125899906842624*a2*l^2*v^2*x*y*cos(theta)^2*cos(z)*sin(z) + 281474976710656*a2*l*v^2*x^2*y*cos(theta)*cos(z)*sin(theta) - 281474976710656*a2*l*v^2*x*y^2*cos(theta)*sin(theta)*sin(z))/(281474976710656*l*v^2*(- sin(z)*x^3 + cos(z)*x^2*y - sin(z)*x*y^2 + 9*sin(z)*x + cos(z)*y^3 + 9*cos(z)*y))];
    
    w1 = [ -(3*(- 3208740581827705672538529988608*v^6*x^2*sin(theta) + 713053462628379038341895553024*v^6*x^4*sin(theta) - 39614081257132168796771975168*v^6*x^6*sin(theta) - 3208740581827705672538529988608*v^6*y^2*sin(theta) - 713053462628379038341895553024*v^6*y^4*sin(theta) - 39614081257132168796771975168*v^6*y^6*sin(theta) + 1508861504564524466226417381849*a0^2*l^4*cos(theta)^4*sin(theta) + 3208740581827705672538529988608*v^6*x^2*cos(theta)^2*sin(theta) - 713053462628379038341895553024*v^6*x^4*cos(theta)^2*sin(theta) + 39614081257132168796771975168*v^6*x^6*cos(theta)^2*sin(theta) - 3208740581827705672538529988608*v^6*y^2*cos(theta)^2*sin(theta) + 6417481163655411345077059977216*v^6*y^2*cos(theta)^4*sin(theta) - 713053462628379038341895553024*v^6*y^4*cos(theta)^2*sin(theta) + 1426106925256758076683791106048*v^6*y^4*cos(theta)^4*sin(theta) - 39614081257132168796771975168*v^6*y^6*cos(theta)^2*sin(theta) + 79228162514264337593543950336*v^6*y^6*cos(theta)^4*sin(theta) - 118842243771396506390315925504*v^6*x^2*y^4*sin(theta) - 118842243771396506390315925504*v^6*x^4*y^2*sin(theta) - 1426106925256758076683791106048*v^6*x^2*y^2*cos(theta)^2*sin(theta) + 1426106925256758076683791106048*v^6*x^2*y^2*cos(theta)^4*sin(theta) - 39614081257132168796771975168*v^6*x^2*y^4*cos(theta)^2*sin(theta) + 39614081257132168796771975168*v^6*x^4*y^2*cos(theta)^2*sin(theta) + 158456325028528675187087900672*v^6*x^2*y^4*cos(theta)^4*sin(theta) + 79228162514264337593543950336*v^6*x^4*y^2*cos(theta)^4*sin(theta) + 38504886981932468070462359863296*l*v^6*y*cos(theta)*cos(z)^3 + 93053476873003464503617369669632*l*v^6*y*cos(theta)^3*cos(z) - 4278320775770274230051373318144*l*v^6*y^3*cos(theta)*cos(z) - 77009773963864936140924719726592*l*v^6*y*cos(theta)^5*cos(z) - 277298568799925181577403826176*l*v^6*y^5*cos(theta)*cos(z) + 22461184072793939707769709920256*l*v^6*x*cos(theta)^3*sin(z) + 4278320775770274230051373318144*l*v^6*x^3*cos(theta)*sin(z) - 198070406285660843983859875840*l*v^6*x^5*cos(theta)*sin(z) - 3802951800684688204490109616128*l^3*v^6*y^3*cos(theta)^3*cos(z)^3 + 5704427701027032306735164424192*l^3*v^6*y^3*cos(theta)^5*cos(z)^3 + 77009773963864936140924719726592*l^2*v^6*cos(theta)^2*cos(z)^2*sin(theta) - 77009773963864936140924719726592*l^2*v^6*cos(theta)^2*cos(z)^4*sin(theta) - 231029321891594808422774159179776*l^2*v^6*cos(theta)^4*cos(z)^2*sin(theta) + 231029321891594808422774159179776*l^2*v^6*cos(theta)^4*cos(z)^4*sin(theta) - 6417481163655411345077059977216*v^6*x^2*cos(theta)^2*cos(z)^2*sin(theta) + 6417481163655411345077059977216*v^6*x^2*cos(theta)^4*cos(z)^2*sin(theta) + 1426106925256758076683791106048*v^6*x^4*cos(theta)^2*cos(z)^2*sin(theta) - 1426106925256758076683791106048*v^6*x^4*cos(theta)^4*cos(z)^2*sin(theta) - 79228162514264337593543950336*v^6*x^6*cos(theta)^2*cos(z)^2*sin(theta) + 79228162514264337593543950336*v^6*x^6*cos(theta)^4*cos(z)^2*sin(theta) + 6417481163655411345077059977216*v^6*y^2*cos(theta)^2*cos(z)^2*sin(theta) - 6417481163655411345077059977216*v^6*y^2*cos(theta)^4*cos(z)^2*sin(theta) + 1426106925256758076683791106048*v^6*y^4*cos(theta)^2*cos(z)^2*sin(theta) - 1426106925256758076683791106048*v^6*y^4*cos(theta)^4*cos(z)^2*sin(theta) + 79228162514264337593543950336*v^6*y^6*cos(theta)^2*cos(z)^2*sin(theta) - 79228162514264337593543950336*v^6*y^6*cos(theta)^4*cos(z)^2*sin(theta) - 115514660945797404211387079589888*l*v^6*y*cos(theta)^3*cos(z)^3 + 8556641551540548460102746636288*l*v^6*y^3*cos(theta)*cos(z)^3 + 21391603878851371150256866590720*l*v^6*y^3*cos(theta)^3*cos(z) + 36365726594047330955436673204224*l^3*v^6*y*cos(theta)^3*cos(z) + 77009773963864936140924719726592*l*v^6*y*cos(theta)^5*cos(z)^3 - 17113283103081096920205493272576*l*v^6*y^3*cos(theta)^5*cos(z) + 475368975085586025561263702016*l*v^6*y^5*cos(theta)*cos(z)^3 + 1228036518971097232699931230208*l*v^6*y^5*cos(theta)^3*cos(z) - 51339849309243290760616479817728*l^3*v^6*y*cos(theta)^5*cos(z) - 950737950171172051122527404032*l*v^6*y^5*cos(theta)^5*cos(z) - 4278320775770274230051373318144*l*v^6*x^3*cos(theta)^3*sin(z) + 2139160387885137115025686659072*l^3*v^6*x*cos(theta)^3*sin(z) + 198070406285660843983859875840*l*v^6*x^5*cos(theta)^3*sin(z) - 16043702909138528362692649943040*l*v^6*y*cos(theta)*cos(z) - 22461184072793939707769709920256*l*v^6*x*cos(theta)*sin(z) + 6417481163655411345077059977216*a2^2*l^4*v^4*cos(theta)^4*sin(theta) + 3111766425056289347504468656128*a0^2*l^4*x^2*cos(theta)^4*sin(theta) + 1431494378410725650296794513408*a0^2*l^4*x^4*cos(theta)^4*sin(theta) - 178263365657094759585473888256*a0^2*l^4*x^6*cos(theta)^4*sin(theta) + 4951760157141521099596496896*a0^2*l^4*x^8*cos(theta)^4*sin(theta) - 3111766425056289347504468656128*a0^2*l^4*y^2*cos(theta)^4*sin(theta) + 1431494378410725650296794513408*a0^2*l^4*y^4*cos(theta)^4*sin(theta) + 178263365657094759585473888256*a0^2*l^4*y^6*cos(theta)^4*sin(theta) + 4951760157141521099596496896*a0^2*l^4*y^8*cos(theta)^4*sin(theta) - 25669924654621645380308239908864*l*v^6*y^3*cos(theta)^3*cos(z)^3 - 34226566206162193840410986545152*l^3*v^6*y*cos(theta)^3*cos(z)^3 + 4040636288227481217270741467136*l^3*v^6*y^3*cos(theta)^3*cos(z) + 17113283103081096920205493272576*l*v^6*y^3*cos(theta)^5*cos(z)^3 - 1426106925256758076683791106048*l*v^6*y^5*cos(theta)^3*cos(z)^3 + 51339849309243290760616479817728*l^3*v^6*y*cos(theta)^5*cos(z)^3 - 5704427701027032306735164424192*l^3*v^6*y^3*cos(theta)^5*cos(z) + 950737950171172051122527404032*l*v^6*y^5*cos(theta)^5*cos(z)^3 - 4278320775770274230051373318144*l^2*v^6*x^2*cos(theta)^2*sin(theta) + 475368975085586025561263702016*l^2*v^6*x^4*cos(theta)^2*sin(theta) - 2139160387885137115025686659072*l^2*v^6*y^2*cos(theta)^2*sin(theta) + 8556641551540548460102746636288*l^2*v^6*y^2*cos(theta)^4*sin(theta) - 237684487542793012780631851008*l^2*v^6*y^4*cos(theta)^2*sin(theta) + 950737950171172051122527404032*l^2*v^6*y^4*cos(theta)^4*sin(theta) + 2852213850513516153367582212096*l^4*v^6*y^2*cos(theta)^4*sin(theta) - 237684487542793012780631851008*l^3*v^6*x^3*cos(theta)^3*sin(z) + 8556641551540548460102746636288*l*v^6*x^2*y*cos(theta)*cos(z)^3 + 18539390028337854996889284378624*l*v^6*x^2*y*cos(theta)^3*cos(z) + 871509787656907713528983453696*l*v^6*x^2*y^3*cos(theta)*cos(z) - 8556641551540548460102746636288*l*v^6*x^2*y*cos(theta)^5*cos(z) - 1426106925256758076683791106048*l*v^6*x^4*y*cos(theta)*cos(z)^3 - 3050284256799176997351442087936*l*v^6*x^4*y*cos(theta)^3*cos(z) + 1901475900342344102245054808064*l*v^6*x^4*y*cos(theta)^5*cos(z) - 4278320775770274230051373318144*a2^2*l^3*v^4*y^3*cos(theta)^3*cos(z)^3 + 5704427701027032306735164424192*a2^2*l^3*v^4*y^3*cos(theta)^5*cos(z)^3 - 237684487542793012780631851008*a2^2*l^3*v^4*y^5*cos(theta)^3*cos(z)^3 + 316912650057057350374175801344*a2^2*l^3*v^4*y^5*cos(theta)^5*cos(z)^3 - 7130534626283790383418955530240*l*v^6*x*y^2*cos(theta)^3*sin(z) + 79228162514264337593543950336*l*v^6*x^3*y^2*cos(theta)*sin(z) + 8556641551540548460102746636288*l*v^6*x*y^2*cos(theta)^5*sin(z) - 1228036518971097232699931230208*l*v^6*x*y^4*cos(theta)^3*sin(z) + 950737950171172051122527404032*l*v^6*x*y^4*cos(theta)^5*sin(z) + 38504886981932468070462359863296*l*v^6*x*cos(theta)*cos(z)^2*sin(z) - 25669924654621645380308239908864*a2^2*l^4*v^4*cos(theta)^4*cos(z)^2*sin(theta) + 25669924654621645380308239908864*a2^2*l^4*v^4*cos(theta)^4*cos(z)^4*sin(theta) + 16043702909138528362692649943040*a2*l*v^5*x*y*cos(theta)^3 - 12834962327310822690154119954432*a2*l*v^5*x*y*cos(theta)^5 + 39614081257132168796771975168*a2*l*v^5*x*y^5*cos(theta) + 39614081257132168796771975168*a2*l*v^5*x^5*y*cos(theta) - 10695801939425685575128433295360*l^2*v^6*x^2*cos(theta)^2*cos(z)^2*sin(theta) + 17113283103081096920205493272576*l^2*v^6*x^2*cos(theta)^2*cos(z)^4*sin(theta) + 42783207757702742300513733181440*l^2*v^6*x^2*cos(theta)^4*cos(z)^2*sin(theta) + 237684487542793012780631851008*l^2*v^6*x^4*cos(theta)^2*cos(z)^2*sin(theta) - 51339849309243290760616479817728*l^2*v^6*x^2*cos(theta)^4*cos(z)^4*sin(theta) - 950737950171172051122527404032*l^2*v^6*x^4*cos(theta)^2*cos(z)^4*sin(theta) - 1901475900342344102245054808064*l^2*v^6*x^4*cos(theta)^4*cos(z)^2*sin(theta) + 2852213850513516153367582212096*l^4*v^6*x^2*cos(theta)^4*cos(z)^2*sin(theta) + 2852213850513516153367582212096*l^2*v^6*x^4*cos(theta)^4*cos(z)^4*sin(theta) + 23530764266736508265282553249792*l^2*v^6*y^2*cos(theta)^2*cos(z)^2*sin(theta) - 17113283103081096920205493272576*l^2*v^6*y^2*cos(theta)^2*cos(z)^4*sin(theta) - 59896490860783839220719226454016*l^2*v^6*y^2*cos(theta)^4*cos(z)^2*sin(theta) + 1663791412799551089464422957056*l^2*v^6*y^4*cos(theta)^2*cos(z)^2*sin(theta) + 51339849309243290760616479817728*l^2*v^6*y^2*cos(theta)^4*cos(z)^4*sin(theta) - 950737950171172051122527404032*l^2*v^6*y^4*cos(theta)^2*cos(z)^4*sin(theta) - 3802951800684688204490109616128*l^2*v^6*y^4*cos(theta)^4*cos(z)^2*sin(theta) - 2852213850513516153367582212096*l^4*v^6*y^2*cos(theta)^4*cos(z)^2*sin(theta) + 2852213850513516153367582212096*l^2*v^6*y^4*cos(theta)^4*cos(z)^4*sin(theta) - 3802951800684688204490109616128*l^3*v^6*x^3*cos(theta)^3*cos(z)^2*sin(z) + 5704427701027032306735164424192*l^3*v^6*x^3*cos(theta)^5*cos(z)^2*sin(z) + 2852213850513516153367582212096*v^6*x^2*y^2*cos(theta)^2*cos(z)^2*sin(theta) - 2852213850513516153367582212096*v^6*x^2*y^2*cos(theta)^4*cos(z)^2*sin(theta) + 79228162514264337593543950336*v^6*x^2*y^4*cos(theta)^2*cos(z)^2*sin(theta) - 79228162514264337593543950336*v^6*x^4*y^2*cos(theta)^2*cos(z)^2*sin(theta) - 79228162514264337593543950336*v^6*x^2*y^4*cos(theta)^4*cos(z)^2*sin(theta) + 79228162514264337593543950336*v^6*x^4*y^2*cos(theta)^4*cos(z)^2*sin(theta) - 396140812571321687967719751680*a0*l^3*v^3*x^3*y^3*cos(theta)^3 + 475368975085586025561263702016*a0*l^3*v^3*x^3*y^3*cos(theta)^5 - 57757330472898702105693539794944*a1*l^3*v^4*y*cos(theta)^3*cos(z)^3 + 12834962327310822690154119954432*a1*l^3*v^4*y^3*cos(theta)^3*cos(z) + 9626221745483117017615589965824*a2^2*l^3*v^4*y*cos(theta)^3*cos(z) + 77009773963864936140924719726592*a1*l^3*v^4*y*cos(theta)^5*cos(z)^3 - 17113283103081096920205493272576*a1*l^3*v^4*y^3*cos(theta)^5*cos(z) + 752667543885511207138667528192*a1*l^3*v^4*y^5*cos(theta)^3*cos(z) - 12834962327310822690154119954432*a2^2*l^3*v^4*y*cos(theta)^5*cos(z) - 950737950171172051122527404032*a1*l^3*v^4*y^5*cos(theta)^5*cos(z) + 3208740581827705672538529988608*a1*l^2*v^4*x^2*cos(theta)^2*sin(theta) - 713053462628379038341895553024*a1*l^2*v^4*x^4*cos(theta)^2*sin(theta) + 39614081257132168796771975168*a1*l^2*v^4*x^6*cos(theta)^2*sin(theta) - 3208740581827705672538529988608*a1*l^2*v^4*y^2*cos(theta)^2*sin(theta) + 12834962327310822690154119954432*a1*l^2*v^4*y^2*cos(theta)^4*sin(theta) - 713053462628379038341895553024*a1*l^2*v^4*y^4*cos(theta)^2*sin(theta) + 2852213850513516153367582212096*a1*l^2*v^4*y^4*cos(theta)^4*sin(theta) - 39614081257132168796771975168*a1*l^2*v^4*y^6*cos(theta)^2*sin(theta) + 8556641551540548460102746636288*a1*l^4*v^4*y^2*cos(theta)^4*sin(theta) + 158456325028528675187087900672*a1*l^2*v^4*y^6*cos(theta)^4*sin(theta) + 950737950171172051122527404032*a1*l^4*v^4*y^4*cos(theta)^4*sin(theta) + 9626221745483117017615589965824*a2^2*l^3*v^4*x*cos(theta)^3*sin(z) - 39614081257132168796771975168*a1*l^3*v^4*x^5*cos(theta)^3*sin(z) - 12834962327310822690154119954432*a2^2*l^3*v^4*x*cos(theta)^5*sin(z) - 24894131400450314780035749249024*a0*l^3*v^3*cos(theta)^3*cos(z)*sin(z) + 37341197100675472170053623873536*a0*l^3*v^3*cos(theta)^5*cos(z)*sin(z) + 51339849309243290760616479817728*a2*l^3*v^5*cos(theta)^3*cos(z)*sin(z) - 77009773963864936140924719726592*a2*l^3*v^5*cos(theta)^5*cos(z)*sin(z) - 25669924654621645380308239908864*l*v^6*x^2*y*cos(theta)^3*cos(z)^3 - 950737950171172051122527404032*l*v^6*x^2*y^3*cos(theta)*cos(z)^3 - 1822247737828079764651510857728*l*v^6*x^2*y^3*cos(theta)^3*cos(z) - 7368219113826583396199587381248*l^3*v^6*x^2*y*cos(theta)^3*cos(z) + 17113283103081096920205493272576*l*v^6*x^2*y*cos(theta)^5*cos(z)^3 + 950737950171172051122527404032*l*v^6*x^2*y^3*cos(theta)^5*cos(z) + 4278320775770274230051373318144*l*v^6*x^4*y*cos(theta)^3*cos(z)^3 + 11408855402054064613470328848384*l^3*v^6*x^2*y*cos(theta)^5*cos(z) - 2852213850513516153367582212096*l*v^6*x^4*y*cos(theta)^5*cos(z)^3 - 1029966112685436388716071354368*l*v^6*x^3*y^2*cos(theta)^3*sin(z) - 4040636288227481217270741467136*l^3*v^6*x*y^2*cos(theta)^3*sin(z) + 950737950171172051122527404032*l*v^6*x^3*y^2*cos(theta)^5*sin(z) + 5704427701027032306735164424192*l^3*v^6*x*y^2*cos(theta)^5*sin(z) - 115514660945797404211387079589888*l*v^6*x*cos(theta)^3*cos(z)^2*sin(z) - 8556641551540548460102746636288*l*v^6*x^3*cos(theta)*cos(z)^2*sin(z) + 77009773963864936140924719726592*l*v^6*x*cos(theta)^5*cos(z)^2*sin(z) + 475368975085586025561263702016*l*v^6*x^5*cos(theta)*cos(z)^2*sin(z) + 5974755181877740648098057682944*a0*l^3*v^3*x*y*cos(theta)^3 - 4149021900075052463339291541504*a0*l^3*v^3*x*y*cos(theta)^5 + 79228162514264337593543950336*a2*l*v^5*x^3*y^3*cos(theta) + 2852213850513516153367582212096*a2*l^3*v^5*x*y*cos(theta)^3 - 198070406285660843983859875840*a2*l*v^5*x*y^5*cos(theta)^3 - 198070406285660843983859875840*a2*l*v^5*x^5*y*cos(theta)^3 + 158456325028528675187087900672*a2*l*v^5*x*y^5*cos(theta)^5 + 158456325028528675187087900672*a2*l*v^5*x^5*y*cos(theta)^5 - 9982748476797306536786537742336*l*v^6*x^2*y*cos(theta)*cos(z) + 1148808356456832895106387279872*l*v^6*x^4*y*cos(theta)*cos(z) - 12834962327310822690154119954432*a1*l^3*v^4*y^3*cos(theta)^3*cos(z)^3 - 19252443490966234035231179931648*a2^2*l^3*v^4*y*cos(theta)^3*cos(z)^3 + 4278320775770274230051373318144*a2^2*l^3*v^4*y^3*cos(theta)^3*cos(z) + 17113283103081096920205493272576*a1*l^3*v^4*y^3*cos(theta)^5*cos(z)^3 - 713053462628379038341895553024*a1*l^3*v^4*y^5*cos(theta)^3*cos(z)^3 + 25669924654621645380308239908864*a2^2*l^3*v^4*y*cos(theta)^5*cos(z)^3 - 5704427701027032306735164424192*a2^2*l^3*v^4*y^3*cos(theta)^5*cos(z) + 356526731314189519170947776512*a2^2*l^3*v^4*y^5*cos(theta)^3*cos(z) + 950737950171172051122527404032*a1*l^3*v^4*y^5*cos(theta)^5*cos(z)^3 - 475368975085586025561263702016*a2^2*l^3*v^4*y^5*cos(theta)^5*cos(z) - 1426106925256758076683791106048*l*v^6*x*y^2*cos(theta)*sin(z) + 277298568799925181577403826176*l*v^6*x*y^4*cos(theta)*sin(z) + 3208740581827705672538529988608*a2^2*l^2*v^4*x^2*cos(theta)^2*sin(theta) - 6417481163655411345077059977216*a2^2*l^2*v^4*x^2*cos(theta)^4*sin(theta) - 713053462628379038341895553024*a2^2*l^2*v^4*x^4*cos(theta)^2*sin(theta) + 1426106925256758076683791106048*a2^2*l^2*v^4*x^4*cos(theta)^4*sin(theta) + 39614081257132168796771975168*a2^2*l^2*v^4*x^6*cos(theta)^2*sin(theta) + 1426106925256758076683791106048*a2^2*l^4*v^4*x^2*cos(theta)^4*sin(theta) - 79228162514264337593543950336*a2^2*l^2*v^4*x^6*cos(theta)^4*sin(theta) + 79228162514264337593543950336*a2^2*l^4*v^4*x^4*cos(theta)^4*sin(theta) + 6417481163655411345077059977216*a1^2*l^4*v^2*y^2*cos(theta)^4*sin(theta) + 1426106925256758076683791106048*a1^2*l^4*v^2*y^4*cos(theta)^4*sin(theta) + 4278320775770274230051373318144*a2^2*l^4*v^4*y^2*cos(theta)^4*sin(theta) + 79228162514264337593543950336*a1^2*l^4*v^2*y^6*cos(theta)^4*sin(theta) + 713053462628379038341895553024*a2^2*l^4*v^4*y^4*cos(theta)^4*sin(theta) - 3554492406833960044483470950400*a0^2*l^4*x^2*y^2*cos(theta)^4*sin(theta) + 178263365657094759585473888256*a0^2*l^4*x^2*y^4*cos(theta)^4*sin(theta) - 178263365657094759585473888256*a0^2*l^4*x^4*y^2*cos(theta)^4*sin(theta) + 19807040628566084398385987584*a0^2*l^4*x^2*y^6*cos(theta)^4*sin(theta) + 29710560942849126597578981376*a0^2*l^4*x^4*y^4*cos(theta)^4*sin(theta) + 19807040628566084398385987584*a0^2*l^4*x^6*y^2*cos(theta)^4*sin(theta) - 118842243771396506390315925504*a2^2*l^3*v^4*x^5*cos(theta)^3*sin(z) + 158456325028528675187087900672*a2^2*l^3*v^4*x^5*cos(theta)^5*sin(z) - 102679698618486581521232959635456*a2*l^3*v^5*cos(theta)^3*cos(z)^3*sin(z) + 154019547927729872281849439453184*a2*l^3*v^5*cos(theta)^5*cos(z)^3*sin(z) + 2852213850513516153367582212096*l*v^6*x^2*y^3*cos(theta)^3*cos(z)^3 + 11408855402054064613470328848384*l^3*v^6*x^2*y*cos(theta)^3*cos(z)^3 - 1901475900342344102245054808064*l*v^6*x^2*y^3*cos(theta)^5*cos(z)^3 - 17113283103081096920205493272576*l^3*v^6*x^2*y*cos(theta)^5*cos(z)^3 - 3208740581827705672538529988608*a2*l*v^5*x*y*cos(theta) + 1188422437713965063903159255040*l^2*v^6*x^2*y^2*cos(theta)^2*sin(theta) - 1901475900342344102245054808064*l^2*v^6*x^2*y^2*cos(theta)^4*sin(theta) + 25669924654621645380308239908864*l*v^6*x^3*cos(theta)^3*cos(z)^2*sin(z) + 34226566206162193840410986545152*l^3*v^6*x*cos(theta)^3*cos(z)^2*sin(z) - 17113283103081096920205493272576*l*v^6*x^3*cos(theta)^5*cos(z)^2*sin(z) - 1426106925256758076683791106048*l*v^6*x^5*cos(theta)^3*cos(z)^2*sin(z) - 51339849309243290760616479817728*l^3*v^6*x*cos(theta)^5*cos(z)^2*sin(z) + 950737950171172051122527404032*l*v^6*x^5*cos(theta)^5*cos(z)^2*sin(z) - 6223532850112578695008937312256*a0*a2*l^4*v^2*cos(theta)^4*sin(theta) - 2852213850513516153367582212096*a0*l^3*v^3*x*y^3*cos(theta)^3 + 2852213850513516153367582212096*a0*l^3*v^3*x^3*y*cos(theta)^3 + 4278320775770274230051373318144*a0*l^3*v^3*x*y^3*cos(theta)^5 - 198070406285660843983859875840*a0*l^3*v^3*x*y^5*cos(theta)^3 - 4278320775770274230051373318144*a0*l^3*v^3*x^3*y*cos(theta)^5 - 198070406285660843983859875840*a0*l^3*v^3*x^5*y*cos(theta)^3 + 237684487542793012780631851008*a0*l^3*v^3*x*y^5*cos(theta)^5 + 237684487542793012780631851008*a0*l^3*v^3*x^5*y*cos(theta)^5 - 396140812571321687967719751680*a2*l*v^5*x^3*y^3*cos(theta)^3 - 2852213850513516153367582212096*a2*l^3*v^5*x*y^3*cos(theta)^3 - 1584563250285286751870879006720*a2*l^3*v^5*x^3*y*cos(theta)^3 + 316912650057057350374175801344*a2*l*v^5*x^3*y^3*cos(theta)^5 + 3802951800684688204490109616128*a2*l^3*v^5*x*y^3*cos(theta)^5 + 1901475900342344102245054808064*a2*l^3*v^5*x^3*y*cos(theta)^5 + 54548589891070996433155009806336*a1*l^3*v^4*y*cos(theta)^3*cos(z) - 77009773963864936140924719726592*a1*l^3*v^4*y*cos(theta)^5*cos(z) + 3208740581827705672538529988608*a1*l^3*v^4*x*cos(theta)^3*sin(z) + 6417481163655411345077059977216*a2*l*v^5*x*y*cos(theta)*cos(z)^2 - 5704427701027032306735164424192*l^2*v^6*x^2*y^2*cos(theta)^2*cos(z)^2*sin(theta) + 5704427701027032306735164424192*l^2*v^6*x^2*y^2*cos(theta)^2*cos(z)^4*sin(theta) + 17113283103081096920205493272576*l^2*v^6*x^2*y^2*cos(theta)^4*cos(z)^2*sin(theta) - 17113283103081096920205493272576*l^2*v^6*x^2*y^2*cos(theta)^4*cos(z)^4*sin(theta) + 12834962327310822690154119954432*v^6*x*y*cos(theta)^2*cos(z)*sin(theta)*sin(z) - 12834962327310822690154119954432*v^6*x*y*cos(theta)^4*cos(z)*sin(theta)*sin(z) + 12447065700225157390017874624512*a0*a2*l^4*v^2*cos(theta)^4*cos(z)^2*sin(theta) + 5704427701027032306735164424192*a0*l^3*v^3*x*y^3*cos(theta)^3*cos(z)^2 - 5704427701027032306735164424192*a0*l^3*v^3*x^3*y*cos(theta)^3*cos(z)^2 - 8556641551540548460102746636288*a0*l^3*v^3*x*y^3*cos(theta)^5*cos(z)^2 + 396140812571321687967719751680*a0*l^3*v^3*x*y^5*cos(theta)^3*cos(z)^2 + 8556641551540548460102746636288*a0*l^3*v^3*x^3*y*cos(theta)^5*cos(z)^2 + 396140812571321687967719751680*a0*l^3*v^3*x^5*y*cos(theta)^3*cos(z)^2 - 12834962327310822690154119954432*a1*l^3*v^4*x^2*y*cos(theta)^3*cos(z)^3 - 633825300114114700748351602688*a1*l^3*v^4*x^2*y^3*cos(theta)^3*cos(z) + 6417481163655411345077059977216*a2^2*l^3*v^4*x^2*y*cos(theta)^3*cos(z) - 475368975085586025561263702016*a0*l^3*v^3*x*y^5*cos(theta)^5*cos(z)^2 - 475368975085586025561263702016*a0*l^3*v^3*x^5*y*cos(theta)^5*cos(z)^2 + 17113283103081096920205493272576*a1*l^3*v^4*x^2*y*cos(theta)^5*cos(z)^3 + 950737950171172051122527404032*a1*l^3*v^4*x^2*y^3*cos(theta)^5*cos(z) + 2139160387885137115025686659072*a1*l^3*v^4*x^4*y*cos(theta)^3*cos(z)^3 + 792281625142643375935439503360*a2*l*v^5*x^3*y^3*cos(theta)^3*cos(z)^2 + 9507379501711720511225274040320*a2*l^3*v^5*x*y^3*cos(theta)^3*cos(z)^2 - 633825300114114700748351602688*a2*l^3*v^5*x^3*y*cos(theta)^3*cos(z)^2 - 8556641551540548460102746636288*a2^2*l^3*v^4*x^2*y*cos(theta)^5*cos(z) - 356526731314189519170947776512*a2^2*l^3*v^4*x^4*y*cos(theta)^3*cos(z) - 2852213850513516153367582212096*a1*l^3*v^4*x^4*y*cos(theta)^5*cos(z)^3 - 633825300114114700748351602688*a2*l*v^5*x^3*y^3*cos(theta)^5*cos(z)^2 - 5070602400912917605986812821504*a2*l^3*v^5*x*y^3*cos(theta)^3*cos(z)^4 - 13310331302396408715715383656448*a2*l^3*v^5*x*y^3*cos(theta)^5*cos(z)^2 + 5070602400912917605986812821504*a2*l^3*v^5*x^3*y*cos(theta)^3*cos(z)^4 + 1901475900342344102245054808064*a2*l^3*v^5*x^3*y*cos(theta)^5*cos(z)^2 + 475368975085586025561263702016*a2^2*l^3*v^4*x^4*y*cos(theta)^5*cos(z) + 7605903601369376408980219232256*a2*l^3*v^5*x*y^3*cos(theta)^5*cos(z)^4 - 7605903601369376408980219232256*a2*l^3*v^5*x^3*y*cos(theta)^5*cos(z)^4 - 1426106925256758076683791106048*a1*l^2*v^4*x^2*y^2*cos(theta)^2*sin(theta) + 2852213850513516153367582212096*a1*l^2*v^4*x^2*y^2*cos(theta)^4*sin(theta) - 39614081257132168796771975168*a1*l^2*v^4*x^2*y^4*cos(theta)^2*sin(theta) + 39614081257132168796771975168*a1*l^2*v^4*x^4*y^2*cos(theta)^2*sin(theta) + 316912650057057350374175801344*a1*l^2*v^4*x^2*y^4*cos(theta)^4*sin(theta) + 158456325028528675187087900672*a1*l^2*v^4*x^4*y^2*cos(theta)^4*sin(theta) + 950737950171172051122527404032*a1*l^4*v^4*x^2*y^2*cos(theta)^4*sin(theta) - 1431494378410725650296794513408*a0*l^2*v^3*x^3*cos(theta)^2*cos(z)*sin(theta) + 5725977513642902601187178053632*a0*l^2*v^3*x^3*cos(theta)^4*cos(z)*sin(theta) + 267395048485642139378210832384*a0*l^2*v^3*x^5*cos(theta)^2*cos(z)*sin(theta) - 1069580193942568557512843329536*a0*l^2*v^3*x^5*cos(theta)^4*cos(z)*sin(theta) - 9903520314283042199192993792*a0*l^2*v^3*x^7*cos(theta)^2*cos(z)*sin(theta) - 4278320775770274230051373318144*a0*l^4*v^3*x^3*cos(theta)^4*cos(z)*sin(theta) - 57757330472898702105693539794944*a2*l^2*v^5*x*cos(theta)^2*cos(z)^3*sin(theta) - 11408855402054064613470328848384*a2*l^2*v^5*x^3*cos(theta)^2*cos(z)*sin(theta) + 39614081257132168796771975168*a0*l^2*v^3*x^7*cos(theta)^4*cos(z)*sin(theta) + 237684487542793012780631851008*a0*l^4*v^3*x^5*cos(theta)^4*cos(z)*sin(theta) + 102679698618486581521232959635456*a2*l^2*v^5*x*cos(theta)^4*cos(z)^3*sin(theta) + 17113283103081096920205493272576*a2*l^2*v^5*x^3*cos(theta)^4*cos(z)*sin(theta) + 594211218856982531951579627520*a2*l^2*v^5*x^5*cos(theta)^2*cos(z)*sin(theta) - 792281625142643375935439503360*a2*l^2*v^5*x^5*cos(theta)^4*cos(z)*sin(theta) - 17113283103081096920205493272576*a2*l^4*v^5*x*cos(theta)^4*cos(z)^3*sin(theta) + 950737950171172051122527404032*a2*l^4*v^5*x^3*cos(theta)^4*cos(z)*sin(theta) - 792281625142643375935439503360*a1*l^3*v^4*x^3*y^2*cos(theta)^3*sin(z) + 2139160387885137115025686659072*a2^2*l^3*v^4*x*y^2*cos(theta)^3*sin(z) + 950737950171172051122527404032*a1*l^3*v^4*x^3*y^2*cos(theta)^5*sin(z) - 2852213850513516153367582212096*a2^2*l^3*v^4*x*y^2*cos(theta)^5*sin(z) - 356526731314189519170947776512*a2^2*l^3*v^4*x*y^4*cos(theta)^3*sin(z) + 475368975085586025561263702016*a2^2*l^3*v^4*x*y^4*cos(theta)^5*sin(z) - 26112650636399316077287242203136*a0*l^3*v^3*x^2*cos(theta)^3*cos(z)*sin(z) + 34355865081857415607123068321792*a0*l^3*v^3*x^2*cos(theta)^5*cos(z)*sin(z) + 4991374238398653268393268871168*a0*l^3*v^3*x^4*cos(theta)^3*cos(z)*sin(z) - 57757330472898702105693539794944*a1*l^3*v^4*x*cos(theta)^3*cos(z)^2*sin(z) - 6417481163655411345077059977216*a0*l^3*v^3*x^4*cos(theta)^5*cos(z)*sin(z) - 198070406285660843983859875840*a0*l^3*v^3*x^6*cos(theta)^3*cos(z)*sin(z) + 77009773963864936140924719726592*a1*l^3*v^4*x*cos(theta)^5*cos(z)^2*sin(z) + 8556641551540548460102746636288*a2*l^3*v^5*x^2*cos(theta)^3*cos(z)*sin(z) + 237684487542793012780631851008*a0*l^3*v^3*x^6*cos(theta)^5*cos(z)*sin(z) - 8556641551540548460102746636288*a2*l^3*v^5*x^2*cos(theta)^5*cos(z)*sin(z) - 1584563250285286751870879006720*a2*l^3*v^5*x^4*cos(theta)^3*cos(z)*sin(z) + 1901475900342344102245054808064*a2*l^3*v^5*x^4*cos(theta)^5*cos(z)*sin(z) + 26112650636399316077287242203136*a0*l^3*v^3*y^2*cos(theta)^3*cos(z)*sin(z) - 34355865081857415607123068321792*a0*l^3*v^3*y^2*cos(theta)^5*cos(z)*sin(z) + 4991374238398653268393268871168*a0*l^3*v^3*y^4*cos(theta)^3*cos(z)*sin(z) - 6417481163655411345077059977216*a0*l^3*v^3*y^4*cos(theta)^5*cos(z)*sin(z) + 198070406285660843983859875840*a0*l^3*v^3*y^6*cos(theta)^3*cos(z)*sin(z) + 31374352355648677687043404333056*a2*l^3*v^5*y^2*cos(theta)^3*cos(z)*sin(z) - 237684487542793012780631851008*a0*l^3*v^3*y^6*cos(theta)^5*cos(z)*sin(z) - 42783207757702742300513733181440*a2*l^3*v^5*y^2*cos(theta)^5*cos(z)*sin(z) + 2852213850513516153367582212096*a2*l^3*v^5*y^4*cos(theta)^3*cos(z)*sin(z) - 3802951800684688204490109616128*a2*l^3*v^5*y^4*cos(theta)^5*cos(z)*sin(z) - 1431494378410725650296794513408*a0*l^2*v^3*y^3*cos(theta)^2*sin(theta)*sin(z) + 5725977513642902601187178053632*a0*l^2*v^3*y^3*cos(theta)^4*sin(theta)*sin(z) - 267395048485642139378210832384*a0*l^2*v^3*y^5*cos(theta)^2*sin(theta)*sin(z) + 1069580193942568557512843329536*a0*l^2*v^3*y^5*cos(theta)^4*sin(theta)*sin(z) - 9903520314283042199192993792*a0*l^2*v^3*y^7*cos(theta)^2*sin(theta)*sin(z) + 4278320775770274230051373318144*a0*l^4*v^3*y^3*cos(theta)^4*sin(theta)*sin(z) - 1426106925256758076683791106048*a2*l^2*v^5*y^3*cos(theta)^2*sin(theta)*sin(z) + 39614081257132168796771975168*a0*l^2*v^3*y^7*cos(theta)^4*sin(theta)*sin(z) + 237684487542793012780631851008*a0*l^4*v^3*y^5*cos(theta)^4*sin(theta)*sin(z) + 5704427701027032306735164424192*a2*l^2*v^5*y^3*cos(theta)^4*sin(theta)*sin(z) - 118842243771396506390315925504*a2*l^2*v^5*y^5*cos(theta)^2*sin(theta)*sin(z) + 475368975085586025561263702016*a2*l^2*v^5*y^5*cos(theta)^4*sin(theta)*sin(z) + 2852213850513516153367582212096*a2*l^4*v^5*y^3*cos(theta)^4*sin(theta)*sin(z) - 118842243771396506390315925504*a1*a2*l^3*v^3*x*y^5*cos(theta)^3 - 118842243771396506390315925504*a1*a2*l^3*v^3*x^5*y*cos(theta)^3 + 158456325028528675187087900672*a1*a2*l^3*v^3*x*y^5*cos(theta)^5 + 158456325028528675187087900672*a1*a2*l^3*v^3*x^5*y*cos(theta)^5 - 4667649637584434021256702984192*a0*a2*l^3*v^2*y*cos(theta)^3*cos(z) + 6223532850112578695008937312256*a0*a2*l^3*v^2*y*cos(theta)^5*cos(z) + 25669924654621645380308239908864*l*v^6*x*y^2*cos(theta)^3*cos(z)^2*sin(z) - 950737950171172051122527404032*l*v^6*x^3*y^2*cos(theta)*cos(z)^2*sin(z) - 17113283103081096920205493272576*l*v^6*x*y^2*cos(theta)^5*cos(z)^2*sin(z) + 4278320775770274230051373318144*l*v^6*x*y^4*cos(theta)^3*cos(z)^2*sin(z) - 2852213850513516153367582212096*l*v^6*x*y^4*cos(theta)^5*cos(z)^2*sin(z) - 4667649637584434021256702984192*a0*a2*l^3*v^2*x*cos(theta)^3*sin(z) + 6223532850112578695008937312256*a0*a2*l^3*v^2*x*cos(theta)^5*sin(z) - 32087405818277056725385299886080*a2*l*v^5*x*y*cos(theta)^3*cos(z)^2 + 25669924654621645380308239908864*a2*l*v^5*x*y*cos(theta)^5*cos(z)^2 - 79228162514264337593543950336*a2*l*v^5*x*y^5*cos(theta)*cos(z)^2 - 79228162514264337593543950336*a2*l*v^5*x^5*y*cos(theta)*cos(z)^2 - 158456325028528675187087900672*v^6*x*y^5*cos(theta)^2*cos(z)*sin(theta)*sin(z) - 158456325028528675187087900672*v^6*x^5*y*cos(theta)^2*cos(z)*sin(theta)*sin(z) + 158456325028528675187087900672*v^6*x*y^5*cos(theta)^4*cos(z)*sin(theta)*sin(z) + 158456325028528675187087900672*v^6*x^5*y*cos(theta)^4*cos(z)*sin(theta)*sin(z) + 3208740581827705672538529988608*a2*l*v^5*x^2*cos(theta)*cos(z)*sin(z) - 713053462628379038341895553024*a2*l*v^5*x^4*cos(theta)*cos(z)*sin(z) + 39614081257132168796771975168*a2*l*v^5*x^6*cos(theta)*cos(z)*sin(z) - 3208740581827705672538529988608*a2*l*v^5*y^2*cos(theta)*cos(z)*sin(z) - 713053462628379038341895553024*a2*l*v^5*y^4*cos(theta)*cos(z)*sin(z) - 39614081257132168796771975168*a2*l*v^5*y^6*cos(theta)*cos(z)*sin(z) + 792281625142643375935439503360*a0*l^3*v^3*x^3*y^3*cos(theta)^3*cos(z)^2 - 950737950171172051122527404032*a0*l^3*v^3*x^3*y^3*cos(theta)^5*cos(z)^2 + 1426106925256758076683791106048*a1*l^3*v^4*x^2*y^3*cos(theta)^3*cos(z)^3 - 4278320775770274230051373318144*a2^2*l^3*v^4*x^2*y*cos(theta)^3*cos(z)^3 - 1901475900342344102245054808064*a1*l^3*v^4*x^2*y^3*cos(theta)^5*cos(z)^3 + 5704427701027032306735164424192*a2^2*l^3*v^4*x^2*y*cos(theta)^5*cos(z)^3 + 713053462628379038341895553024*a2^2*l^3*v^4*x^4*y*cos(theta)^3*cos(z)^3 - 950737950171172051122527404032*a2^2*l^3*v^4*x^4*y*cos(theta)^5*cos(z)^3 - 713053462628379038341895553024*a2^2*l^2*v^4*x^2*y^2*cos(theta)^2*sin(theta) + 1426106925256758076683791106048*a1^2*l^4*v^2*x^2*y^2*cos(theta)^4*sin(theta) + 1426106925256758076683791106048*a2^2*l^2*v^4*x^2*y^2*cos(theta)^4*sin(theta) + 39614081257132168796771975168*a2^2*l^2*v^4*x^2*y^4*cos(theta)^2*sin(theta) + 79228162514264337593543950336*a2^2*l^2*v^4*x^4*y^2*cos(theta)^2*sin(theta) + 158456325028528675187087900672*a1^2*l^4*v^2*x^2*y^4*cos(theta)^4*sin(theta) + 79228162514264337593543950336*a1^2*l^4*v^2*x^4*y^2*cos(theta)^4*sin(theta) - 79228162514264337593543950336*a2^2*l^2*v^4*x^2*y^4*cos(theta)^4*sin(theta) - 158456325028528675187087900672*a2^2*l^2*v^4*x^4*y^2*cos(theta)^4*sin(theta) + 475368975085586025561263702016*a2^2*l^4*v^4*x^2*y^2*cos(theta)^4*sin(theta) - 6417481163655411345077059977216*a1*l^2*v^4*x^2*cos(theta)^2*cos(z)^2*sin(theta) + 12834962327310822690154119954432*a1*l^2*v^4*x^2*cos(theta)^4*cos(z)^2*sin(theta) + 1426106925256758076683791106048*a1*l^2*v^4*x^4*cos(theta)^2*cos(z)^2*sin(theta) - 2852213850513516153367582212096*a1*l^2*v^4*x^4*cos(theta)^4*cos(z)^2*sin(theta) - 79228162514264337593543950336*a1*l^2*v^4*x^6*cos(theta)^2*cos(z)^2*sin(theta) - 8556641551540548460102746636288*a1*l^4*v^4*x^2*cos(theta)^4*cos(z)^2*sin(theta) + 12834962327310822690154119954432*a2*l^2*v^5*x^3*cos(theta)^2*cos(z)^3*sin(theta) + 158456325028528675187087900672*a1*l^2*v^4*x^6*cos(theta)^4*cos(z)^2*sin(theta) + 950737950171172051122527404032*a1*l^4*v^4*x^4*cos(theta)^4*cos(z)^2*sin(theta) - 22817710804108129226940657696768*a2*l^2*v^5*x^3*cos(theta)^4*cos(z)^3*sin(theta) - 713053462628379038341895553024*a2*l^2*v^5*x^5*cos(theta)^2*cos(z)^3*sin(theta) + 1267650600228229401496703205376*a2*l^2*v^5*x^5*cos(theta)^4*cos(z)^3*sin(theta) + 1901475900342344102245054808064*a2*l^4*v^5*x^3*cos(theta)^4*cos(z)^3*sin(theta) - 475368975085586025561263702016*a2^2*l^3*v^4*x^3*y^2*cos(theta)^3*sin(z) + 633825300114114700748351602688*a2^2*l^3*v^4*x^3*y^2*cos(theta)^5*sin(z) + 6417481163655411345077059977216*a1*l^2*v^4*y^2*cos(theta)^2*cos(z)^2*sin(theta) - 12834962327310822690154119954432*a1*l^2*v^4*y^2*cos(theta)^4*cos(z)^2*sin(theta) + 1426106925256758076683791106048*a1*l^2*v^4*y^4*cos(theta)^2*cos(z)^2*sin(theta) - 2852213850513516153367582212096*a1*l^2*v^4*y^4*cos(theta)^4*cos(z)^2*sin(theta) + 79228162514264337593543950336*a1*l^2*v^4*y^6*cos(theta)^2*cos(z)^2*sin(theta) - 8556641551540548460102746636288*a1*l^4*v^4*y^2*cos(theta)^4*cos(z)^2*sin(theta) - 158456325028528675187087900672*a1*l^2*v^4*y^6*cos(theta)^4*cos(z)^2*sin(theta) - 950737950171172051122527404032*a1*l^4*v^4*y^4*cos(theta)^4*cos(z)^2*sin(theta) + 12834962327310822690154119954432*a1*l^3*v^4*x^3*cos(theta)^3*cos(z)^2*sin(z) - 19252443490966234035231179931648*a2^2*l^3*v^4*x*cos(theta)^3*cos(z)^2*sin(z) - 17113283103081096920205493272576*a1*l^3*v^4*x^3*cos(theta)^5*cos(z)^2*sin(z) - 713053462628379038341895553024*a1*l^3*v^4*x^5*cos(theta)^3*cos(z)^2*sin(z) + 22817710804108129226940657696768*a2*l^3*v^5*x^2*cos(theta)^3*cos(z)^3*sin(z) + 25669924654621645380308239908864*a2^2*l^3*v^4*x*cos(theta)^5*cos(z)^2*sin(z) + 950737950171172051122527404032*a1*l^3*v^4*x^5*cos(theta)^5*cos(z)^2*sin(z) - 34226566206162193840410986545152*a2*l^3*v^5*x^2*cos(theta)^5*cos(z)^3*sin(z) - 1267650600228229401496703205376*a2*l^3*v^5*x^4*cos(theta)^3*cos(z)^3*sin(z) + 1901475900342344102245054808064*a2*l^3*v^5*x^4*cos(theta)^5*cos(z)^3*sin(z) - 22817710804108129226940657696768*a2*l^3*v^5*y^2*cos(theta)^3*cos(z)^3*sin(z) + 34226566206162193840410986545152*a2*l^3*v^5*y^2*cos(theta)^5*cos(z)^3*sin(z) - 1267650600228229401496703205376*a2*l^3*v^5*y^4*cos(theta)^3*cos(z)^3*sin(z) + 1901475900342344102245054808064*a2*l^3*v^5*y^4*cos(theta)^5*cos(z)^3*sin(z) - 237684487542793012780631851008*a1*a2*l^3*v^3*x^3*y^3*cos(theta)^3 + 316912650057057350374175801344*a1*a2*l^3*v^3*x^3*y^3*cos(theta)^5 + 4294483135232176950890383540224*a0*a2*l^3*v^2*y^3*cos(theta)^3*cos(z) - 5725977513642902601187178053632*a0*a2*l^3*v^2*y^3*cos(theta)^5*cos(z) + 802185145456926418134632497152*a0*a2*l^3*v^2*y^5*cos(theta)^3*cos(z) - 1069580193942568557512843329536*a0*a2*l^3*v^2*y^5*cos(theta)^5*cos(z) + 29710560942849126597578981376*a0*a2*l^3*v^2*y^7*cos(theta)^3*cos(z) - 39614081257132168796771975168*a0*a2*l^3*v^2*y^7*cos(theta)^5*cos(z) + 2852213850513516153367582212096*l*v^6*x^3*y^2*cos(theta)^3*cos(z)^2*sin(z) + 11408855402054064613470328848384*l^3*v^6*x*y^2*cos(theta)^3*cos(z)^2*sin(z) - 1901475900342344102245054808064*l*v^6*x^3*y^2*cos(theta)^5*cos(z)^2*sin(z) - 17113283103081096920205493272576*l^3*v^6*x*y^2*cos(theta)^5*cos(z)^2*sin(z) - 7108984813667920088966941900800*a0*a2*l^4*v^2*x^2*cos(theta)^4*sin(theta) - 356526731314189519170947776512*a0*a2*l^4*v^2*x^4*cos(theta)^4*sin(theta) + 39614081257132168796771975168*a0*a2*l^4*v^2*x^6*cos(theta)^4*sin(theta) + 4342970213617885113407414206464*a0*a2*l^4*v^2*y^2*cos(theta)^4*sin(theta) + 2495687119199326634196634435584*a0*a2*l^4*v^2*y^4*cos(theta)^4*sin(theta) + 118842243771396506390315925504*a0*a2*l^4*v^2*y^6*cos(theta)^4*sin(theta) - 4294483135232176950890383540224*a0*a2*l^3*v^2*x^3*cos(theta)^3*sin(z) + 5725977513642902601187178053632*a0*a2*l^3*v^2*x^3*cos(theta)^5*sin(z) + 802185145456926418134632497152*a0*a2*l^3*v^2*x^5*cos(theta)^3*sin(z) - 1069580193942568557512843329536*a0*a2*l^3*v^2*x^5*cos(theta)^5*sin(z) - 29710560942849126597578981376*a0*a2*l^3*v^2*x^7*cos(theta)^3*sin(z) + 39614081257132168796771975168*a0*a2*l^3*v^2*x^7*cos(theta)^5*sin(z) - 11949510363755481296196115365888*a0*l^3*v^3*x*y*cos(theta)^3*cos(z)^2 + 8298043800150104926678583083008*a0*l^3*v^3*x*y*cos(theta)^5*cos(z)^2 + 7843588088912169421760851083264*a1*l^3*v^4*x^2*y*cos(theta)^3*cos(z) - 8556641551540548460102746636288*a1*l^3*v^4*x^2*y*cos(theta)^5*cos(z) - 1386492843999625907887019130880*a1*l^3*v^4*x^4*y*cos(theta)^3*cos(z) - 158456325028528675187087900672*a2*l*v^5*x^3*y^3*cos(theta)*cos(z)^2 + 45635421608216258453881315393536*a2*l^3*v^5*x*y*cos(theta)^3*cos(z)^2 + 1901475900342344102245054808064*a1*l^3*v^4*x^4*y*cos(theta)^5*cos(z) + 396140812571321687967719751680*a2*l*v^5*x*y^5*cos(theta)^3*cos(z)^2 + 396140812571321687967719751680*a2*l*v^5*x^5*y*cos(theta)^3*cos(z)^2 - 45635421608216258453881315393536*a2*l^3*v^5*x*y*cos(theta)^3*cos(z)^4 - 68453132412324387680821973090304*a2*l^3*v^5*x*y*cos(theta)^5*cos(z)^2 - 316912650057057350374175801344*a2*l*v^5*x*y^5*cos(theta)^5*cos(z)^2 - 316912650057057350374175801344*a2*l*v^5*x^5*y*cos(theta)^5*cos(z)^2 + 68453132412324387680821973090304*a2*l^3*v^5*x*y*cos(theta)^5*cos(z)^4 - 316912650057057350374175801344*v^6*x^3*y^3*cos(theta)^2*cos(z)*sin(theta)*sin(z) + 316912650057057350374175801344*v^6*x^3*y^3*cos(theta)^4*cos(z)*sin(theta)*sin(z) - 1555883212528144673752234328064*a0*l^2*v^3*x*cos(theta)^2*cos(z)*sin(theta) + 6223532850112578695008937312256*a0*l^2*v^3*x*cos(theta)^4*cos(z)*sin(theta) - 4149021900075052463339291541504*a0*l^4*v^3*x*cos(theta)^4*cos(z)*sin(theta) + 54548589891070996433155009806336*a2*l^2*v^5*x*cos(theta)^2*cos(z)*sin(theta) - 89844736291175758831078839681024*a2*l^2*v^5*x*cos(theta)^4*cos(z)*sin(theta) + 8556641551540548460102746636288*a2*l^4*v^5*x*cos(theta)^4*cos(z)*sin(theta) - 4991374238398653268393268871168*a1*l^3*v^4*x*y^2*cos(theta)^3*sin(z) + 8556641551540548460102746636288*a1*l^3*v^4*x*y^2*cos(theta)^5*sin(z) - 752667543885511207138667528192*a1*l^3*v^4*x*y^4*cos(theta)^3*sin(z) + 950737950171172051122527404032*a1*l^3*v^4*x*y^4*cos(theta)^5*sin(z) - 16043702909138528362692649943040*a2*l*v^5*x^2*cos(theta)^3*cos(z)*sin(z) + 12834962327310822690154119954432*a2*l*v^5*x^2*cos(theta)^5*cos(z)*sin(z) + 3565267313141895191709477765120*a2*l*v^5*x^4*cos(theta)^3*cos(z)*sin(z) - 2852213850513516153367582212096*a2*l*v^5*x^4*cos(theta)^5*cos(z)*sin(z) - 198070406285660843983859875840*a2*l*v^5*x^6*cos(theta)^3*cos(z)*sin(z) + 158456325028528675187087900672*a2*l*v^5*x^6*cos(theta)^5*cos(z)*sin(z) + 16043702909138528362692649943040*a2*l*v^5*y^2*cos(theta)^3*cos(z)*sin(z) - 12834962327310822690154119954432*a2*l*v^5*y^2*cos(theta)^5*cos(z)*sin(z) + 3565267313141895191709477765120*a2*l*v^5*y^4*cos(theta)^3*cos(z)*sin(z) - 2852213850513516153367582212096*a2*l*v^5*y^4*cos(theta)^5*cos(z)*sin(z) + 198070406285660843983859875840*a2*l*v^5*y^6*cos(theta)^3*cos(z)*sin(z) - 158456325028528675187087900672*a2*l*v^5*y^6*cos(theta)^5*cos(z)*sin(z) + 475368975085586025561263702016*a2^2*l^3*v^4*x^2*y^3*cos(theta)^3*cos(z)^3 - 633825300114114700748351602688*a2^2*l^3*v^4*x^2*y^3*cos(theta)^5*cos(z)^3 + 1555883212528144673752234328064*a0*l^2*v^3*y*cos(theta)^2*sin(theta)*sin(z) - 6223532850112578695008937312256*a0*l^2*v^3*y*cos(theta)^4*sin(theta)*sin(z) - 4149021900075052463339291541504*a0*l^4*v^3*y*cos(theta)^4*sin(theta)*sin(z) - 3208740581827705672538529988608*a2*l^2*v^5*y*cos(theta)^2*sin(theta)*sin(z) + 12834962327310822690154119954432*a2*l^2*v^5*y*cos(theta)^4*sin(theta)*sin(z) + 8556641551540548460102746636288*a2*l^4*v^5*y*cos(theta)^4*sin(theta)*sin(z) + 9626221745483117017615589965824*a1*a2*l^3*v^3*x*y*cos(theta)^3 - 12834962327310822690154119954432*a1*a2*l^3*v^3*x*y*cos(theta)^5 - 8556641551540548460102746636288*l*v^6*x*y^2*cos(theta)*cos(z)^2*sin(z) - 1426106925256758076683791106048*l*v^6*x*y^4*cos(theta)*cos(z)^2*sin(z) - 3208740581827705672538529988608*a2^2*l^2*v^4*x^2*cos(theta)^2*cos(z)^2*sin(theta) + 6417481163655411345077059977216*a1^2*l^4*v^2*x^2*cos(theta)^4*cos(z)^2*sin(theta) + 6417481163655411345077059977216*a2^2*l^2*v^4*x^2*cos(theta)^4*cos(z)^2*sin(theta) + 713053462628379038341895553024*a2^2*l^2*v^4*x^4*cos(theta)^2*cos(z)^2*sin(theta) - 1426106925256758076683791106048*a1^2*l^4*v^2*x^4*cos(theta)^4*cos(z)^2*sin(theta) - 1426106925256758076683791106048*a2^2*l^2*v^4*x^4*cos(theta)^4*cos(z)^2*sin(theta) - 39614081257132168796771975168*a2^2*l^2*v^4*x^6*cos(theta)^2*cos(z)^2*sin(theta) + 79228162514264337593543950336*a1^2*l^4*v^2*x^6*cos(theta)^4*cos(z)^2*sin(theta) + 79228162514264337593543950336*a2^2*l^2*v^4*x^6*cos(theta)^4*cos(z)^2*sin(theta) - 5704427701027032306735164424192*a2^2*l^4*v^4*x^2*cos(theta)^4*cos(z)^4*sin(theta) + 316912650057057350374175801344*a2^2*l^4*v^4*x^4*cos(theta)^4*cos(z)^2*sin(theta) + 316912650057057350374175801344*a2^2*l^4*v^4*x^4*cos(theta)^4*cos(z)^4*sin(theta) + 3208740581827705672538529988608*a2^2*l^2*v^4*y^2*cos(theta)^2*cos(z)^2*sin(theta) - 6417481163655411345077059977216*a1^2*l^4*v^2*y^2*cos(theta)^4*cos(z)^2*sin(theta) - 6417481163655411345077059977216*a2^2*l^2*v^4*y^2*cos(theta)^4*cos(z)^2*sin(theta) + 713053462628379038341895553024*a2^2*l^2*v^4*y^4*cos(theta)^2*cos(z)^2*sin(theta) - 1426106925256758076683791106048*a1^2*l^4*v^2*y^4*cos(theta)^4*cos(z)^2*sin(theta) - 1426106925256758076683791106048*a2^2*l^2*v^4*y^4*cos(theta)^4*cos(z)^2*sin(theta) + 39614081257132168796771975168*a2^2*l^2*v^4*y^6*cos(theta)^2*cos(z)^2*sin(theta) - 11408855402054064613470328848384*a2^2*l^4*v^4*y^2*cos(theta)^4*cos(z)^2*sin(theta) - 79228162514264337593543950336*a1^2*l^4*v^2*y^6*cos(theta)^4*cos(z)^2*sin(theta) - 79228162514264337593543950336*a2^2*l^2*v^4*y^6*cos(theta)^4*cos(z)^2*sin(theta) + 5704427701027032306735164424192*a2^2*l^4*v^4*y^2*cos(theta)^4*cos(z)^4*sin(theta) - 950737950171172051122527404032*a2^2*l^4*v^4*y^4*cos(theta)^4*cos(z)^2*sin(theta) + 316912650057057350374175801344*a2^2*l^4*v^4*y^4*cos(theta)^4*cos(z)^4*sin(theta) + 4278320775770274230051373318144*a2^2*l^3*v^4*x^3*cos(theta)^3*cos(z)^2*sin(z) - 5704427701027032306735164424192*a2^2*l^3*v^4*x^3*cos(theta)^5*cos(z)^2*sin(z) - 237684487542793012780631851008*a2^2*l^3*v^4*x^5*cos(theta)^3*cos(z)^2*sin(z) + 316912650057057350374175801344*a2^2*l^3*v^4*x^5*cos(theta)^5*cos(z)^2*sin(z) + 178263365657094759585473888256*a0*l^2*v^3*x^3*y^2*cos(theta)^2*cos(z)*sin(theta) - 713053462628379038341895553024*a0*l^2*v^3*x^3*y^2*cos(theta)^4*cos(z)*sin(theta) - 29710560942849126597578981376*a0*l^2*v^3*x^3*y^4*cos(theta)^2*cos(z)*sin(theta) - 29710560942849126597578981376*a0*l^2*v^3*x^5*y^2*cos(theta)^2*cos(z)*sin(theta) + 118842243771396506390315925504*a0*l^2*v^3*x^3*y^4*cos(theta)^4*cos(z)*sin(theta) + 118842243771396506390315925504*a0*l^2*v^3*x^5*y^2*cos(theta)^4*cos(z)*sin(theta) + 475368975085586025561263702016*a0*l^4*v^3*x^3*y^2*cos(theta)^4*cos(z)*sin(theta) + 12834962327310822690154119954432*a2*l^2*v^5*x*y^2*cos(theta)^2*cos(z)^3*sin(theta) - 950737950171172051122527404032*a2*l^2*v^5*x^3*y^2*cos(theta)^2*cos(z)*sin(theta) - 22817710804108129226940657696768*a2*l^2*v^5*x*y^2*cos(theta)^4*cos(z)^3*sin(theta) + 2139160387885137115025686659072*a2*l^2*v^5*x*y^4*cos(theta)^2*cos(z)^3*sin(theta) + 2218388550399401452619230609408*a2*l^2*v^5*x^3*y^2*cos(theta)^4*cos(z)*sin(theta) - 3802951800684688204490109616128*a2*l^2*v^5*x*y^4*cos(theta)^4*cos(z)^3*sin(theta) - 5704427701027032306735164424192*a2*l^4*v^5*x*y^2*cos(theta)^4*cos(z)^3*sin(theta) - 1426106925256758076683791106048*a0*l^3*v^3*x^2*y^2*cos(theta)^3*cos(z)*sin(z) + 4278320775770274230051373318144*a0*l^3*v^3*x^2*y^2*cos(theta)^5*cos(z)*sin(z) + 198070406285660843983859875840*a0*l^3*v^3*x^2*y^4*cos(theta)^3*cos(z)*sin(z) - 198070406285660843983859875840*a0*l^3*v^3*x^4*y^2*cos(theta)^3*cos(z)*sin(z) + 12834962327310822690154119954432*a1*l^3*v^4*x*y^2*cos(theta)^3*cos(z)^2*sin(z) - 237684487542793012780631851008*a0*l^3*v^3*x^2*y^4*cos(theta)^5*cos(z)*sin(z) + 237684487542793012780631851008*a0*l^3*v^3*x^4*y^2*cos(theta)^5*cos(z)*sin(z) - 17113283103081096920205493272576*a1*l^3*v^4*x*y^2*cos(theta)^5*cos(z)^2*sin(z) + 2139160387885137115025686659072*a1*l^3*v^4*x*y^4*cos(theta)^3*cos(z)^2*sin(z) - 3802951800684688204490109616128*a2*l^3*v^5*x^2*y^2*cos(theta)^3*cos(z)*sin(z) - 2852213850513516153367582212096*a1*l^3*v^4*x*y^4*cos(theta)^5*cos(z)^2*sin(z) + 5704427701027032306735164424192*a2*l^3*v^5*x^2*y^2*cos(theta)^5*cos(z)*sin(z) - 178263365657094759585473888256*a0*l^2*v^3*x^2*y^3*cos(theta)^2*sin(theta)*sin(z) + 713053462628379038341895553024*a0*l^2*v^3*x^2*y^3*cos(theta)^4*sin(theta)*sin(z) - 29710560942849126597578981376*a0*l^2*v^3*x^2*y^5*cos(theta)^2*sin(theta)*sin(z) - 29710560942849126597578981376*a0*l^2*v^3*x^4*y^3*cos(theta)^2*sin(theta)*sin(z) + 118842243771396506390315925504*a0*l^2*v^3*x^2*y^5*cos(theta)^4*sin(theta)*sin(z) + 118842243771396506390315925504*a0*l^2*v^3*x^4*y^3*cos(theta)^4*sin(theta)*sin(z) + 475368975085586025561263702016*a0*l^4*v^3*x^2*y^3*cos(theta)^4*sin(theta)*sin(z) + 475368975085586025561263702016*a2*l^2*v^5*x^2*y^3*cos(theta)^2*sin(theta)*sin(z) - 316912650057057350374175801344*a2*l^2*v^5*x^2*y^3*cos(theta)^4*sin(theta)*sin(z) + 57757330472898702105693539794944*a2*l^2*v^5*y*cos(theta)^2*cos(z)^2*sin(theta)*sin(z) - 102679698618486581521232959635456*a2*l^2*v^5*y*cos(theta)^4*cos(z)^2*sin(theta)*sin(z) - 17113283103081096920205493272576*a2*l^4*v^5*y*cos(theta)^4*cos(z)^2*sin(theta)*sin(z) - 5331738610250940066725206425600*a0*a2*l^3*v^2*x^2*y*cos(theta)^3*cos(z) + 7108984813667920088966941900800*a0*a2*l^3*v^2*x^2*y*cos(theta)^5*cos(z) - 267395048485642139378210832384*a0*a2*l^3*v^2*x^4*y*cos(theta)^3*cos(z) - 19252443490966234035231179931648*a1*a2*l^3*v^3*x*y*cos(theta)^3*cos(z)^2 + 356526731314189519170947776512*a0*a2*l^3*v^2*x^4*y*cos(theta)^5*cos(z) + 29710560942849126597578981376*a0*a2*l^3*v^2*x^6*y*cos(theta)^3*cos(z) + 25669924654621645380308239908864*a1*a2*l^3*v^3*x*y*cos(theta)^5*cos(z)^2 - 39614081257132168796771975168*a0*a2*l^3*v^2*x^6*y*cos(theta)^5*cos(z) + 5725977513642902601187178053632*a0*a1*l^4*v*x^3*cos(theta)^4*cos(z)*sin(theta) - 1069580193942568557512843329536*a0*a1*l^4*v*x^5*cos(theta)^4*cos(z)*sin(theta) - 12834962327310822690154119954432*a1*a2*l^4*v^3*x*cos(theta)^4*cos(z)*sin(theta) + 39614081257132168796771975168*a0*a1*l^4*v*x^7*cos(theta)^4*cos(z)*sin(theta) + 5331738610250940066725206425600*a0*a2*l^3*v^2*x*y^2*cos(theta)^3*sin(z) - 7108984813667920088966941900800*a0*a2*l^3*v^2*x*y^2*cos(theta)^5*sin(z) - 267395048485642139378210832384*a0*a2*l^3*v^2*x*y^4*cos(theta)^3*sin(z) + 356526731314189519170947776512*a0*a2*l^3*v^2*x*y^4*cos(theta)^5*sin(z) - 29710560942849126597578981376*a0*a2*l^3*v^2*x*y^6*cos(theta)^3*sin(z) + 39614081257132168796771975168*a0*a2*l^3*v^2*x*y^6*cos(theta)^5*sin(z) + 34226566206162193840410986545152*l^2*v^6*x*y*cos(theta)^2*cos(z)^3*sin(theta)*sin(z) - 3327582825599102178928845914112*l^2*v^6*x*y^3*cos(theta)^2*cos(z)*sin(theta)*sin(z) + 475368975085586025561263702016*l^2*v^6*x^3*y*cos(theta)^2*cos(z)*sin(theta)*sin(z) - 102679698618486581521232959635456*l^2*v^6*x*y*cos(theta)^4*cos(z)^3*sin(theta)*sin(z) + 7605903601369376408980219232256*l^2*v^6*x*y^3*cos(theta)^4*cos(z)*sin(theta)*sin(z) - 3802951800684688204490109616128*l^2*v^6*x^3*y*cos(theta)^4*cos(z)*sin(theta)*sin(z) + 5725977513642902601187178053632*a0*a1*l^4*v*y^3*cos(theta)^4*sin(theta)*sin(z) + 1069580193942568557512843329536*a0*a1*l^4*v*y^5*cos(theta)^4*sin(theta)*sin(z) + 12834962327310822690154119954432*a1*a2*l^4*v^3*y*cos(theta)^4*sin(theta)*sin(z) + 39614081257132168796771975168*a0*a1*l^4*v*y^7*cos(theta)^4*sin(theta)*sin(z) - 1426106925256758076683791106048*a2*l*v^5*x^2*y^2*cos(theta)*cos(z)*sin(z) - 39614081257132168796771975168*a2*l*v^5*x^2*y^4*cos(theta)*cos(z)*sin(z) + 39614081257132168796771975168*a2*l*v^5*x^4*y^2*cos(theta)*cos(z)*sin(z) + 2852213850513516153367582212096*a1*l^2*v^4*x^2*y^2*cos(theta)^2*cos(z)^2*sin(theta) - 5704427701027032306735164424192*a1*l^2*v^4*x^2*y^2*cos(theta)^4*cos(z)^2*sin(theta) + 79228162514264337593543950336*a1*l^2*v^4*x^2*y^4*cos(theta)^2*cos(z)^2*sin(theta) - 79228162514264337593543950336*a1*l^2*v^4*x^4*y^2*cos(theta)^2*cos(z)^2*sin(theta) - 158456325028528675187087900672*a1*l^2*v^4*x^2*y^4*cos(theta)^4*cos(z)^2*sin(theta) + 158456325028528675187087900672*a1*l^2*v^4*x^4*y^2*cos(theta)^4*cos(z)^2*sin(theta) + 1426106925256758076683791106048*a2*l^2*v^5*x^3*y^2*cos(theta)^2*cos(z)^3*sin(theta) - 2535301200456458802993406410752*a2*l^2*v^5*x^3*y^2*cos(theta)^4*cos(z)^3*sin(theta) + 1426106925256758076683791106048*a1*l^3*v^4*x^3*y^2*cos(theta)^3*cos(z)^2*sin(z) + 4278320775770274230051373318144*a2^2*l^3*v^4*x*y^2*cos(theta)^3*cos(z)^2*sin(z) - 1901475900342344102245054808064*a1*l^3*v^4*x^3*y^2*cos(theta)^5*cos(z)^2*sin(z) + 7605903601369376408980219232256*a2*l^3*v^5*x^2*y^2*cos(theta)^3*cos(z)^3*sin(z) - 5704427701027032306735164424192*a2^2*l^3*v^4*x*y^2*cos(theta)^5*cos(z)^2*sin(z) + 713053462628379038341895553024*a2^2*l^3*v^4*x*y^4*cos(theta)^3*cos(z)^2*sin(z) - 11408855402054064613470328848384*a2*l^3*v^5*x^2*y^2*cos(theta)^5*cos(z)^3*sin(z) - 950737950171172051122527404032*a2^2*l^3*v^4*x*y^4*cos(theta)^5*cos(z)^2*sin(z) + 12834962327310822690154119954432*a2*l^2*v^5*y^3*cos(theta)^2*cos(z)^2*sin(theta)*sin(z) - 22817710804108129226940657696768*a2*l^2*v^5*y^3*cos(theta)^4*cos(z)^2*sin(theta)*sin(z) + 713053462628379038341895553024*a2*l^2*v^5*y^5*cos(theta)^2*cos(z)^2*sin(theta)*sin(z) - 1267650600228229401496703205376*a2*l^2*v^5*y^5*cos(theta)^4*cos(z)^2*sin(theta)*sin(z) - 1901475900342344102245054808064*a2*l^4*v^5*y^3*cos(theta)^4*cos(z)^2*sin(theta)*sin(z) + 534790096971284278756421664768*a0*a2*l^3*v^2*x^2*y^3*cos(theta)^3*cos(z) - 713053462628379038341895553024*a0*a2*l^3*v^2*x^2*y^3*cos(theta)^5*cos(z) + 89131682828547379792736944128*a0*a2*l^3*v^2*x^2*y^5*cos(theta)^3*cos(z) + 89131682828547379792736944128*a0*a2*l^3*v^2*x^4*y^3*cos(theta)^3*cos(z) - 118842243771396506390315925504*a0*a2*l^3*v^2*x^2*y^5*cos(theta)^5*cos(z) - 118842243771396506390315925504*a0*a2*l^3*v^2*x^4*y^3*cos(theta)^5*cos(z) + 237684487542793012780631851008*a1*a2*l^3*v^3*x*y^5*cos(theta)^3*cos(z)^2 + 237684487542793012780631851008*a1*a2*l^3*v^3*x^5*y*cos(theta)^3*cos(z)^2 - 316912650057057350374175801344*a1*a2*l^3*v^3*x*y^5*cos(theta)^5*cos(z)^2 - 316912650057057350374175801344*a1*a2*l^3*v^3*x^5*y*cos(theta)^5*cos(z)^2 - 713053462628379038341895553024*a0*a2*l^4*v^2*x^2*y^2*cos(theta)^4*sin(theta) + 277298568799925181577403826176*a0*a2*l^4*v^2*x^2*y^4*cos(theta)^4*sin(theta) + 198070406285660843983859875840*a0*a2*l^4*v^2*x^4*y^2*cos(theta)^4*sin(theta) + 25669924654621645380308239908864*a1*a2*l^4*v^3*x*cos(theta)^4*cos(z)^3*sin(theta) + 158456325028528675187087900672*a1*a2*l^4*v^3*x^5*cos(theta)^4*cos(z)*sin(theta) + 534790096971284278756421664768*a0*a2*l^3*v^2*x^3*y^2*cos(theta)^3*sin(z) - 713053462628379038341895553024*a0*a2*l^3*v^2*x^3*y^2*cos(theta)^5*sin(z) - 89131682828547379792736944128*a0*a2*l^3*v^2*x^3*y^4*cos(theta)^3*sin(z) - 89131682828547379792736944128*a0*a2*l^3*v^2*x^5*y^2*cos(theta)^3*sin(z) + 118842243771396506390315925504*a0*a2*l^3*v^2*x^3*y^4*cos(theta)^5*sin(z) + 118842243771396506390315925504*a0*a2*l^3*v^2*x^5*y^2*cos(theta)^5*sin(z) + 3802951800684688204490109616128*l^2*v^6*x*y^3*cos(theta)^2*cos(z)^3*sin(theta)*sin(z) - 3802951800684688204490109616128*l^2*v^6*x^3*y*cos(theta)^2*cos(z)^3*sin(theta)*sin(z) - 11408855402054064613470328848384*l^2*v^6*x*y^3*cos(theta)^4*cos(z)^3*sin(theta)*sin(z) + 11408855402054064613470328848384*l^2*v^6*x^3*y*cos(theta)^4*cos(z)^3*sin(theta)*sin(z) - 9626221745483117017615589965824*a1*a2*l^3*v^3*x^2*cos(theta)^3*cos(z)*sin(z) + 12834962327310822690154119954432*a1*a2*l^3*v^3*x^2*cos(theta)^5*cos(z)*sin(z) + 2139160387885137115025686659072*a1*a2*l^3*v^3*x^4*cos(theta)^3*cos(z)*sin(z) - 2852213850513516153367582212096*a1*a2*l^3*v^3*x^4*cos(theta)^5*cos(z)*sin(z) - 118842243771396506390315925504*a1*a2*l^3*v^3*x^6*cos(theta)^3*cos(z)*sin(z) + 158456325028528675187087900672*a1*a2*l^3*v^3*x^6*cos(theta)^5*cos(z)*sin(z) + 9626221745483117017615589965824*a1*a2*l^3*v^3*y^2*cos(theta)^3*cos(z)*sin(z) - 12834962327310822690154119954432*a1*a2*l^3*v^3*y^2*cos(theta)^5*cos(z)*sin(z) + 2139160387885137115025686659072*a1*a2*l^3*v^3*y^4*cos(theta)^3*cos(z)*sin(z) - 2852213850513516153367582212096*a1*a2*l^3*v^3*y^4*cos(theta)^5*cos(z)*sin(z) + 118842243771396506390315925504*a1*a2*l^3*v^3*y^6*cos(theta)^3*cos(z)*sin(z) - 158456325028528675187087900672*a1*a2*l^3*v^3*y^6*cos(theta)^5*cos(z)*sin(z) + 5704427701027032306735164424192*a1*a2*l^4*v^3*y^3*cos(theta)^4*sin(theta)*sin(z) + 475368975085586025561263702016*a1*a2*l^4*v^3*y^5*cos(theta)^4*sin(theta)*sin(z) + 1777246203416980022241735475200*a0*l^2*v^3*x*y^2*cos(theta)^2*cos(z)*sin(theta) - 7108984813667920088966941900800*a0*l^2*v^3*x*y^2*cos(theta)^4*cos(z)*sin(theta) - 89131682828547379792736944128*a0*l^2*v^3*x*y^4*cos(theta)^2*cos(z)*sin(theta) + 356526731314189519170947776512*a0*l^2*v^3*x*y^4*cos(theta)^4*cos(z)*sin(theta) - 9903520314283042199192993792*a0*l^2*v^3*x*y^6*cos(theta)^2*cos(z)*sin(theta) + 4278320775770274230051373318144*a0*l^4*v^3*x*y^2*cos(theta)^4*cos(z)*sin(theta) - 6417481163655411345077059977216*a2*l^2*v^5*x*y^2*cos(theta)^2*cos(z)*sin(theta) + 39614081257132168796771975168*a0*l^2*v^3*x*y^6*cos(theta)^4*cos(z)*sin(theta) + 237684487542793012780631851008*a0*l^4*v^3*x*y^4*cos(theta)^4*cos(z)*sin(theta) + 11408855402054064613470328848384*a2*l^2*v^5*x*y^2*cos(theta)^4*cos(z)*sin(theta) - 1544949169028154583074107031552*a2*l^2*v^5*x*y^4*cos(theta)^2*cos(z)*sin(theta) + 3010670175542044828554670112768*a2*l^2*v^5*x*y^4*cos(theta)^4*cos(z)*sin(theta) + 6655165651198204357857691828224*a2*l^4*v^5*x*y^2*cos(theta)^4*cos(z)*sin(theta) + 7130534626283790383418955530240*a2*l*v^5*x^2*y^2*cos(theta)^3*cos(z)*sin(z) - 5704427701027032306735164424192*a2*l*v^5*x^2*y^2*cos(theta)^5*cos(z)*sin(z) + 198070406285660843983859875840*a2*l*v^5*x^2*y^4*cos(theta)^3*cos(z)*sin(z) - 198070406285660843983859875840*a2*l*v^5*x^4*y^2*cos(theta)^3*cos(z)*sin(z) - 158456325028528675187087900672*a2*l*v^5*x^2*y^4*cos(theta)^5*cos(z)*sin(z) + 158456325028528675187087900672*a2*l*v^5*x^4*y^2*cos(theta)^5*cos(z)*sin(z) + 1777246203416980022241735475200*a0*l^2*v^3*x^2*y*cos(theta)^2*sin(theta)*sin(z) - 7108984813667920088966941900800*a0*l^2*v^3*x^2*y*cos(theta)^4*sin(theta)*sin(z) + 89131682828547379792736944128*a0*l^2*v^3*x^4*y*cos(theta)^2*sin(theta)*sin(z) - 356526731314189519170947776512*a0*l^2*v^3*x^4*y*cos(theta)^4*sin(theta)*sin(z) - 9903520314283042199192993792*a0*l^2*v^3*x^6*y*cos(theta)^2*sin(theta)*sin(z) - 4278320775770274230051373318144*a0*l^4*v^3*x^2*y*cos(theta)^4*sin(theta)*sin(z) - 6417481163655411345077059977216*a2*l^2*v^5*x^2*y*cos(theta)^2*sin(theta)*sin(z) + 39614081257132168796771975168*a0*l^2*v^3*x^6*y*cos(theta)^4*sin(theta)*sin(z) + 237684487542793012780631851008*a0*l^4*v^3*x^4*y*cos(theta)^4*sin(theta)*sin(z) + 11408855402054064613470328848384*a2*l^2*v^5*x^2*y*cos(theta)^4*sin(theta)*sin(z) + 594211218856982531951579627520*a2*l^2*v^5*x^4*y*cos(theta)^2*sin(theta)*sin(z) - 792281625142643375935439503360*a2*l^2*v^5*x^4*y*cos(theta)^4*sin(theta)*sin(z) + 950737950171172051122527404032*a2*l^4*v^5*x^2*y*cos(theta)^4*sin(theta)*sin(z) + 1426106925256758076683791106048*a2^2*l^2*v^4*x^2*y^2*cos(theta)^2*cos(z)^2*sin(theta) - 2852213850513516153367582212096*a1^2*l^4*v^2*x^2*y^2*cos(theta)^4*cos(z)^2*sin(theta) - 2852213850513516153367582212096*a2^2*l^2*v^4*x^2*y^2*cos(theta)^4*cos(z)^2*sin(theta) + 39614081257132168796771975168*a2^2*l^2*v^4*x^2*y^4*cos(theta)^2*cos(z)^2*sin(theta) - 39614081257132168796771975168*a2^2*l^2*v^4*x^4*y^2*cos(theta)^2*cos(z)^2*sin(theta) - 79228162514264337593543950336*a1^2*l^4*v^2*x^2*y^4*cos(theta)^4*cos(z)^2*sin(theta) + 79228162514264337593543950336*a1^2*l^4*v^2*x^4*y^2*cos(theta)^4*cos(z)^2*sin(theta) - 79228162514264337593543950336*a2^2*l^2*v^4*x^2*y^4*cos(theta)^4*cos(z)^2*sin(theta) + 79228162514264337593543950336*a2^2*l^2*v^4*x^4*y^2*cos(theta)^4*cos(z)^2*sin(theta) + 1901475900342344102245054808064*a2^2*l^4*v^4*x^2*y^2*cos(theta)^4*cos(z)^2*sin(theta) - 1901475900342344102245054808064*a2^2*l^4*v^4*x^2*y^2*cos(theta)^4*cos(z)^4*sin(theta) + 475368975085586025561263702016*a2^2*l^3*v^4*x^3*y^2*cos(theta)^3*cos(z)^2*sin(z) - 633825300114114700748351602688*a2^2*l^3*v^4*x^3*y^2*cos(theta)^5*cos(z)^2*sin(z) + 6223532850112578695008937312256*a0*a1*l^4*v*x*cos(theta)^4*cos(z)*sin(theta) - 17113283103081096920205493272576*l^2*v^6*x*y*cos(theta)^2*cos(z)*sin(theta)*sin(z) + 51339849309243290760616479817728*l^2*v^6*x*y*cos(theta)^4*cos(z)*sin(theta)*sin(z) + 5704427701027032306735164424192*l^4*v^6*x*y*cos(theta)^4*cos(z)*sin(theta)*sin(z) + 475368975085586025561263702016*a1*a2*l^3*v^3*x^3*y^3*cos(theta)^3*cos(z)^2 - 633825300114114700748351602688*a1*a2*l^3*v^3*x^3*y^3*cos(theta)^5*cos(z)^2 - 6223532850112578695008937312256*a0*a1*l^4*v*y*cos(theta)^4*sin(theta)*sin(z) + 11451955027285805202374356107264*a0*a2*l^4*v^2*x^2*cos(theta)^4*cos(z)^2*sin(theta) - 2139160387885137115025686659072*a0*a2*l^4*v^2*x^4*cos(theta)^4*cos(z)^2*sin(theta) + 79228162514264337593543950336*a0*a2*l^4*v^2*x^6*cos(theta)^4*cos(z)^2*sin(theta) - 5704427701027032306735164424192*a1*a2*l^4*v^3*x^3*cos(theta)^4*cos(z)^3*sin(theta) + 316912650057057350374175801344*a1*a2*l^4*v^3*x^5*cos(theta)^4*cos(z)^3*sin(theta) - 11451955027285805202374356107264*a0*a2*l^4*v^2*y^2*cos(theta)^4*cos(z)^2*sin(theta) - 2139160387885137115025686659072*a0*a2*l^4*v^2*y^4*cos(theta)^4*cos(z)^2*sin(theta) - 79228162514264337593543950336*a0*a2*l^4*v^2*y^6*cos(theta)^4*cos(z)^2*sin(theta) - 713053462628379038341895553024*a0*a1*l^4*v*x^3*y^2*cos(theta)^4*cos(z)*sin(theta) + 118842243771396506390315925504*a0*a1*l^4*v*x^3*y^4*cos(theta)^4*cos(z)*sin(theta) + 118842243771396506390315925504*a0*a1*l^4*v*x^5*y^2*cos(theta)^4*cos(z)*sin(theta) + 2852213850513516153367582212096*a1*a2*l^4*v^3*x*y^2*cos(theta)^4*cos(z)*sin(theta) + 1109194275199700726309615304704*a1*a2*l^4*v^3*x*y^4*cos(theta)^4*cos(z)*sin(theta) + 713053462628379038341895553024*a0*a1*l^4*v*x^2*y^3*cos(theta)^4*sin(theta)*sin(z) + 118842243771396506390315925504*a0*a1*l^4*v*x^2*y^5*cos(theta)^4*sin(theta)*sin(z) + 118842243771396506390315925504*a0*a1*l^4*v*x^4*y^3*cos(theta)^4*sin(theta)*sin(z) + 2852213850513516153367582212096*a1*a2*l^4*v^3*x^2*y*cos(theta)^4*sin(theta)*sin(z) + 158456325028528675187087900672*a1*a2*l^4*v^3*x^4*y*cos(theta)^4*sin(theta)*sin(z) + 12834962327310822690154119954432*a1*l^2*v^4*x*y*cos(theta)^2*cos(z)*sin(theta)*sin(z) - 25669924654621645380308239908864*a1*l^2*v^4*x*y*cos(theta)^4*cos(z)*sin(theta)*sin(z) - 1426106925256758076683791106048*a2*l^2*v^5*x^2*y^3*cos(theta)^2*cos(z)^2*sin(theta)*sin(z) - 158456325028528675187087900672*a2^2*l^2*v^4*x^3*y^3*cos(theta)^2*cos(z)*sin(theta)*sin(z) + 316912650057057350374175801344*a1^2*l^4*v^2*x^3*y^3*cos(theta)^4*cos(z)*sin(theta)*sin(z) + 2535301200456458802993406410752*a2*l^2*v^5*x^2*y^3*cos(theta)^4*cos(z)^2*sin(theta)*sin(z) + 316912650057057350374175801344*a2^2*l^2*v^4*x^3*y^3*cos(theta)^4*cos(z)*sin(theta)*sin(z) - 1267650600228229401496703205376*a2^2*l^4*v^4*x*y^3*cos(theta)^4*cos(z)^3*sin(theta)*sin(z) + 1267650600228229401496703205376*a2^2*l^4*v^4*x^3*y*cos(theta)^4*cos(z)^3*sin(theta)*sin(z) - 5704427701027032306735164424192*a1*a2*l^4*v^3*x*y^2*cos(theta)^4*cos(z)^3*sin(theta) + 1267650600228229401496703205376*a1*a2*l^4*v^3*x^3*y^2*cos(theta)^4*cos(z)*sin(theta) - 950737950171172051122527404032*a1*a2*l^4*v^3*x*y^4*cos(theta)^4*cos(z)^3*sin(theta) + 4278320775770274230051373318144*a1*a2*l^3*v^3*x^2*y^2*cos(theta)^3*cos(z)*sin(z) - 5704427701027032306735164424192*a1*a2*l^3*v^3*x^2*y^2*cos(theta)^5*cos(z)*sin(z) + 118842243771396506390315925504*a1*a2*l^3*v^3*x^2*y^4*cos(theta)^3*cos(z)*sin(z) - 118842243771396506390315925504*a1*a2*l^3*v^3*x^4*y^2*cos(theta)^3*cos(z)*sin(z) - 158456325028528675187087900672*a1*a2*l^3*v^3*x^2*y^4*cos(theta)^5*cos(z)*sin(z) + 158456325028528675187087900672*a1*a2*l^3*v^3*x^4*y^2*cos(theta)^5*cos(z)*sin(z) + 633825300114114700748351602688*a1*a2*l^4*v^3*x^2*y^3*cos(theta)^4*sin(theta)*sin(z) - 25669924654621645380308239908864*a1*a2*l^4*v^3*y*cos(theta)^4*cos(z)^2*sin(theta)*sin(z) + 6417481163655411345077059977216*a2^2*l^2*v^4*x*y*cos(theta)^2*cos(z)*sin(theta)*sin(z) - 12834962327310822690154119954432*a1^2*l^4*v^2*x*y*cos(theta)^4*cos(z)*sin(theta)*sin(z) - 158456325028528675187087900672*a1*l^2*v^4*x*y^5*cos(theta)^2*cos(z)*sin(theta)*sin(z) - 158456325028528675187087900672*a1*l^2*v^4*x^5*y*cos(theta)^2*cos(z)*sin(theta)*sin(z) - 12834962327310822690154119954432*a2^2*l^2*v^4*x*y*cos(theta)^4*cos(z)*sin(theta)*sin(z) + 316912650057057350374175801344*a1*l^2*v^4*x*y^5*cos(theta)^4*cos(z)*sin(theta)*sin(z) + 316912650057057350374175801344*a1*l^2*v^4*x^5*y*cos(theta)^4*cos(z)*sin(theta)*sin(z) + 1901475900342344102245054808064*a1*l^4*v^4*x*y^3*cos(theta)^4*cos(z)*sin(theta)*sin(z) + 1901475900342344102245054808064*a1*l^4*v^4*x^3*y*cos(theta)^4*cos(z)*sin(theta)*sin(z) + 5704427701027032306735164424192*a2^2*l^4*v^4*x*y*cos(theta)^4*cos(z)*sin(theta)*sin(z) - 7108984813667920088966941900800*a0*a1*l^4*v*x*y^2*cos(theta)^4*cos(z)*sin(theta) + 356526731314189519170947776512*a0*a1*l^4*v*x*y^4*cos(theta)^4*cos(z)*sin(theta) + 39614081257132168796771975168*a0*a1*l^4*v*x*y^6*cos(theta)^4*cos(z)*sin(theta) - 7108984813667920088966941900800*a0*a1*l^4*v*x^2*y*cos(theta)^4*sin(theta)*sin(z) - 356526731314189519170947776512*a0*a1*l^4*v*x^4*y*cos(theta)^4*sin(theta)*sin(z) + 39614081257132168796771975168*a0*a1*l^4*v*x^6*y*cos(theta)^4*sin(theta)*sin(z) + 1426106925256758076683791106048*a0*a2*l^4*v^2*x^2*y^2*cos(theta)^4*cos(z)^2*sin(theta) - 79228162514264337593543950336*a0*a2*l^4*v^2*x^2*y^4*cos(theta)^4*cos(z)^2*sin(theta) + 79228162514264337593543950336*a0*a2*l^4*v^2*x^4*y^2*cos(theta)^4*cos(z)^2*sin(theta) - 633825300114114700748351602688*a1*a2*l^4*v^3*x^3*y^2*cos(theta)^4*cos(z)^3*sin(theta) - 5704427701027032306735164424192*a1*a2*l^4*v^3*y^3*cos(theta)^4*cos(z)^2*sin(theta)*sin(z) - 316912650057057350374175801344*a1*a2*l^4*v^3*y^5*cos(theta)^4*cos(z)^2*sin(theta)*sin(z) - 316912650057057350374175801344*a1*l^2*v^4*x^3*y^3*cos(theta)^2*cos(z)*sin(theta)*sin(z) + 12834962327310822690154119954432*a2*l^2*v^5*x^2*y*cos(theta)^2*cos(z)^2*sin(theta)*sin(z) + 633825300114114700748351602688*a1*l^2*v^4*x^3*y^3*cos(theta)^4*cos(z)*sin(theta)*sin(z) - 22817710804108129226940657696768*a2*l^2*v^5*x^2*y*cos(theta)^4*cos(z)^2*sin(theta)*sin(z) - 2139160387885137115025686659072*a2*l^2*v^5*x^4*y*cos(theta)^2*cos(z)^2*sin(theta)*sin(z) - 79228162514264337593543950336*a2^2*l^2*v^4*x*y^5*cos(theta)^2*cos(z)*sin(theta)*sin(z) - 79228162514264337593543950336*a2^2*l^2*v^4*x^5*y*cos(theta)^2*cos(z)*sin(theta)*sin(z) + 158456325028528675187087900672*a1^2*l^4*v^2*x*y^5*cos(theta)^4*cos(z)*sin(theta)*sin(z) + 158456325028528675187087900672*a1^2*l^4*v^2*x^5*y*cos(theta)^4*cos(z)*sin(theta)*sin(z) + 3802951800684688204490109616128*a2*l^2*v^5*x^4*y*cos(theta)^4*cos(z)^2*sin(theta)*sin(z) + 5704427701027032306735164424192*a2*l^4*v^5*x^2*y*cos(theta)^4*cos(z)^2*sin(theta)*sin(z) + 158456325028528675187087900672*a2^2*l^2*v^4*x*y^5*cos(theta)^4*cos(z)*sin(theta)*sin(z) + 158456325028528675187087900672*a2^2*l^2*v^4*x^5*y*cos(theta)^4*cos(z)*sin(theta)*sin(z) - 11408855402054064613470328848384*a2^2*l^4*v^4*x*y*cos(theta)^4*cos(z)^3*sin(theta)*sin(z) + 1901475900342344102245054808064*a2^2*l^4*v^4*x*y^3*cos(theta)^4*cos(z)*sin(theta)*sin(z) + 633825300114114700748351602688*a2^2*l^4*v^4*x^3*y*cos(theta)^4*cos(z)*sin(theta)*sin(z) + 316912650057057350374175801344*a0*a2*l^4*v^2*x^3*y^3*cos(theta)^4*cos(z)*sin(theta)*sin(z) - 5704427701027032306735164424192*a1*a2*l^4*v^3*x^2*y*cos(theta)^4*cos(z)^2*sin(theta)*sin(z) + 950737950171172051122527404032*a1*a2*l^4*v^3*x^4*y*cos(theta)^4*cos(z)^2*sin(theta)*sin(z) - 2766014600050034975559527694336*a0*a2*l^4*v^2*x*y*cos(theta)^4*cos(z)*sin(theta)*sin(z) + 633825300114114700748351602688*a1*a2*l^4*v^3*x^2*y^3*cos(theta)^4*cos(z)^2*sin(theta)*sin(z) + 2852213850513516153367582212096*a0*a2*l^4*v^2*x*y^3*cos(theta)^4*cos(z)*sin(theta)*sin(z) - 2852213850513516153367582212096*a0*a2*l^4*v^2*x^3*y*cos(theta)^4*cos(z)*sin(theta)*sin(z) + 158456325028528675187087900672*a0*a2*l^4*v^2*x*y^5*cos(theta)^4*cos(z)*sin(theta)*sin(z) + 158456325028528675187087900672*a0*a2*l^4*v^2*x^5*y*cos(theta)^4*cos(z)*sin(theta)*sin(z)))/(79228162514264337593543950336*l^2*v^4*cos(theta)*(3*x^2*y^4 + 3*x^4*y^2 - 81*x^2*cos(2*z) + 18*x^4*cos(2*z) - x^6*cos(2*z) + 81*y^2*cos(2*z) + 18*y^4*cos(2*z) + y^6*cos(2*z) + 81*x^2 - 18*x^4 + x^6 + 81*y^2 + 18*y^4 + y^6 + 36*x^2*y^2*cos(2*z) + x^2*y^4*cos(2*z) - x^4*y^2*cos(2*z) - 4*x^3*y^3*sin(2*z) + 162*x*y*sin(2*z) - 2*x*y^5*sin(2*z) - 2*x^5*y*sin(2*z)));
